simulink model "TwoSpeed_harness"  (Simulink 7.7)
settings: Solver=ode3  SolverMode=SingleTasking  StartTime=0.0  StopTime=100  FixedStep=.0005  RelTol=1e-3
PostLoadFcn:
  | cd '..';
  | PostLoadFcn;
  | cd 'harness';
InitFcn:
  | if signalbuilder('TwoSpeed_harness/Signal_Builder','activegroup') == 1
  |   CD_TWOSPEED_FUNCTION.DataType = 'uint8';
  |   CD_TWOSPEED_FUNCTION.Value = 255;
  | else
  |   CD_TWOSPEED_FUNCTION.DataType = 'uint8';
  |   CD_TWOSPEED_FUNCTION.Value = 0;
  | end
  | 
  | if signalbuilder('TwoSpeed_harness/Signal_Builder','activegroup') == 3
  |   CD_AUTOSHIFT_FUNCTION.DataType = 'uint8';
  |   CD_AUTOSHIFT_FUNCTION.Value = 0;
  |   CD_TWOSPEED_SWITCH_SOURCE.DataType = 'uint8';
  |   CD_TWOSPEED_SWITCH_SOURCE.Value = 23;
  | elseif signalbuilder('TwoSpeed_harness/Signal_Builder','activegroup') == 4
  |   CD_AUTOSHIFT_FUNCTION.DataType = 'uint8';
  |   CD_AUTOSHIFT_FUNCTION.Value = 0;
  |   CD_AUTOSHIFT_TRAVEL_DELAY.DataType = 'uint8';
  |   CD_AUTOSHIFT_TRAVEL_DELAY.Value = 0;
  | else
  |   CD_AUTOSHIFT_FUNCTION.DataType = 'uint8';
  |   CD_AUTOSHIFT_FUNCTION.Value = 255;
  |   CD_TWOSPEED_SWITCH_SOURCE.DataType = 'uint8';
  |   CD_TWOSPEED_SWITCH_SOURCE.Value = 176;
  |   CD_AUTOSHIFT_TRAVEL_DELAY.DataType = 'uint8';
  |   CD_AUTOSHIFT_TRAVEL_DELAY.Value = 32;
  | end
undefined symbols (not defined in the file): ACTIVE, CD_AUTOSHIFT_PHIGH1, CD_AUTOSHIFT_PHIGH2, CD_AUTOSHIFT_PHIGH_TEMP1, CD_AUTOSHIFT_PHIGH_TEMP2, CD_AUTOSHIFT_PLOW1, CD_AUTOSHIFT_PLOW2, CD_AUTOSHIFT_PLOW_TEMP1, CD_AUTOSHIFT_PLOW_TEMP2, CD_PRECISION_REF_NOMINAL_VALUE, CD_TWOSPEED_AFBK_GAIN, CD_TWOSPEED_DEBOUNCE_OPEN_CIRCUIT, CD_TWOSPEED_DEBOUNCE_SHORT_TO_BATTERY, CD_TWOSPEED_DEBOUNCE_SHORT_TO_GROUND, CD_VBATTERY_FILTER_DISPLAY_GAIN, CD_VBATTERY_FILTER_GAIN, CD_VBATTERY_GAIN, ENGINE_CRANKING, EXTREMELY_HIGH, FULL_ON, HIGH, INACTIVE, LOW, NON_FUNCTIONAL, NORMAL, OORH, OORL, SA_GATEWAY, sigbuilder_block, srate, srate100, SYS_NORMAL
libraries: simulink x12, MX_Library x1
settings Model: Creator=smindema  LastModifiedBy=aliebel  CovPath=Aux_Hydraulics/Aux_Hydraulics  CovMetricSettings=dcmw  CovHTMLOptions=-aTS=1 -bRG=1 -bTC=1 -hTR=0 -nFC=0 -scm=1 -bcm=1 -xEv=0  covSaveCumulativeToWorkspaceVar=off  CovSaveSingleToWorkspaceVar=off
settings MATStruct: SampleTime=0.01  Offset=0  Priority=[1.0]
settings DataIOCC: LimitDataPoints=off  SaveOutput=off  SaveTime=off
settings OptimizationCC: BlockReduction=off  InlineParams=on  ExpressionFolding=off  StateBitsets=on  DataBitsets=on  UseTempVars=on  InitFltsAndDblsToZero=on  NoFixptDivByZeroProtection=on  EfficientFloat2IntCast=on  OptimizeModelRefInitCode=on
settings DebuggingCC: SaveWithParameterizedLinksMsg=none  MultiTaskDSMMsg=warning  MultiTaskCondExecSysMsg=none  IntegerOverflowMsg=none  ModelReferenceCSMismatchMessage=warning
settings HardwareCC: ProdBitPerInt=16  ProdBitPerPointer=16  ProdIntDivRoundTo=Floor  ProdEndianess=BigEndian  ProdWordSize=16  ProdHWDeviceType=Motorola HC12
settings ModelReferenceCC: ModelReferenceNumInstancesAllowed=Single
settings RTWCC: SystemTargetFile=ert.tlc  GenCodeOnly=on  TemplateMakefile=ert_default_tmf  Description=Real-Time Workshop Embedded Coder (no auto configuration)  GenerateReport=on  RetainRTWFile=on  ProcessScript=ert_make_rtw_hook  IncludeHyperlinkInReport=on  LaunchReport=on  IncludeERTFirstTime=on
settings RTWCC: CustomHeaderCode=|
  | #include "cpp_req_defines.h"
  | #include "hw_fin.h"
  | #include "cdata.h"
settings CodeAppCC: IgnoreCustomStorageClasses=off  DefineNamingRule=UpperCase
settings ERTTargetCC: TargetFcnLib=ansi_tfl_tmw.mat  FunctionExecutionProfile=off  MultiwordLength=2048  GenerateSampleERTMain=on  IncludeMdlTerminateFcn=off  SupportAbsoluteTime=off  SupportNonFinite=off  SupportComplex=off  PurelyIntegerCode=on  ERTCustomFileTemplate=gen_rtw_req_defines_h.tlc  GlobalDataDefinition=InSeparateSourceFile  GlobalDataReference=InSeparateHeaderFile  ConvertIfToSwitch=off

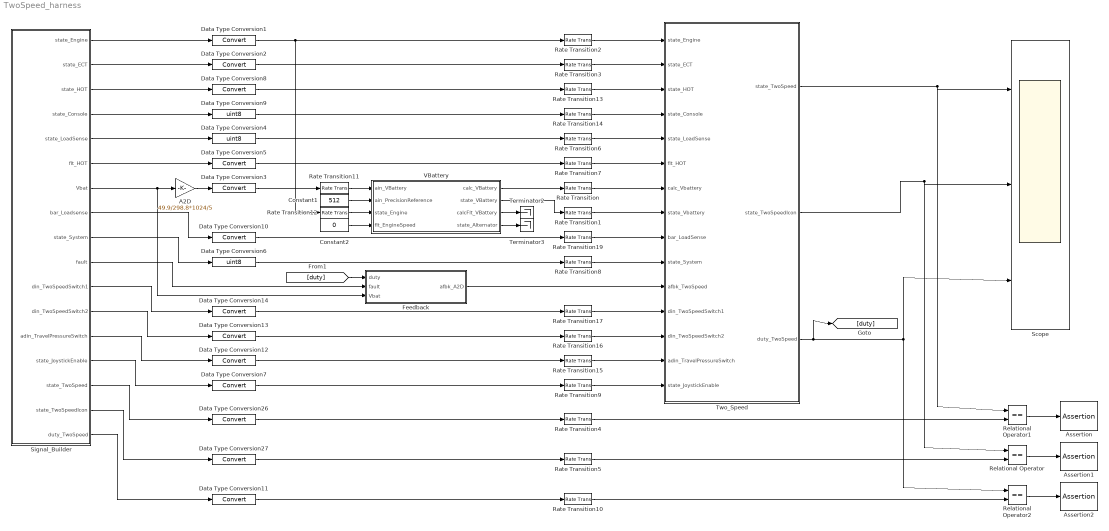
== system TwoSpeed_harness ==
  A2D : Gain  Gain=49.9/298.8*1024/5  OutDataTypeStr=uint16
  Assertion : Assertion  Enabled=off
  Assertion1 : Assertion  Enabled=off
  Assertion2 : Assertion  Enabled=off
  Constant1 : Constant  Value=512  OutDataTypeStr=uint16
  Constant2 : Constant  Value=0  OutDataTypeStr=uint16
  Data Type Conversion{1..3,5,7..8,10..14,26..27} (13 alike) : DataTypeConversion
  Data Type Conversion4 : DataTypeConversion  OutDataTypeStr=uint8
  Data Type Conversion6 : DataTypeConversion  OutDataTypeStr=uint8
  Data Type Conversion9 : DataTypeConversion  OutDataTypeStr=uint8
  Feedback : Subsystem
  Rate Transition : RateTransition  X0=12
  Rate Transition1 : RateTransition  X0=8
  Rate Transition{2..17,19} (17 alike) : RateTransition
  Relational Operator : RelationalOperator  Operator===  OutDataTypeStr=boolean
  Relational Operator1 : RelationalOperator  Operator===  OutDataTypeStr=boolean
  Relational Operator2 : RelationalOperator  Operator===  OutDataTypeStr=boolean
  Scope : Scope  NumInputPorts=3
      settings: TimeRange=50  YMin=0~0~0  YMax=0.3~1~1.25  DataFormat=Array
  Signal_Builder : Subsystem  Tag=STV Subsys  LoadFcn=sigbuilder_block('load');  StartFcn=sigbuilder_block('start');  StopFcn=sigbuilder_block('stop');  ClipboardFcn=sigbuilder_block('clipboard');  mask(Sigbuilder block){}
      mask help: Sigbuilder GUI
      mask init:
      | if ~strcmp(get_param(bdroot(gcbh),'SimulationStatus'),'stopped') tuvar = sigbuilder_block('maskInit'); end
      settings: CopyFcn=sigbuilder_block('copy');  DeleteFcn=sigbuilder_block('delete');  ModelCloseFcn=sigbuilder_block('modelClose');  PreSaveFcn=sigbuilder_block('preSave');  NameChangeFcn=sigbuilder_block('namechange');  OpenFcn=sigbuilder_block('open',[202.5 108.75 780.75 697.5 ]);  CloseFcn=sigbuilder_block('close');
      mask Display: plot(0,0,100,100,[10,10,40,40,10],[80,20,20,80,80],[40,10],[50,50], [40,27,10],[65,72,56],[40,25,25,10],[28,28,43,43]);
  Terminator2 : Terminator
  Terminator3 : Terminator
  Two_Speed : Subsystem  TreatAsAtomicUnit=on  SystemSampleTime=srate  RTWFileName=mod_Outputs
      settings: RTWSystemCode=Function  RTWFcnNameOpts=Use subsystem name  RTWFileNameOpts=User specified
  VBattery : Subsystem  TreatAsAtomicUnit=on  SystemSampleTime=srate100  RTWFileName=mod_Inputs
      settings: RTWSystemCode=Function  RTWFcnNameOpts=Use subsystem name  RTWFileNameOpts=User specified
  wires:
  Signal_Builder/2(state_ECT) -> Data Type Conversion2/1
  Relational Operator/1 -> Assertion1/1
  Signal_Builder/1(state_Engine) -> Data Type Conversion1/1
  Signal_Builder/5(state_LoadSense) -> Data Type Conversion4/1
  Relational Operator1/1 -> Assertion/1
  Data Type Conversion26/1 -> Rate Transition4/1
  Data Type Conversion27/1 -> Rate Transition5/1
  Data Type Conversion1/1 -> Rate Transition2/1, Rate Transition12/1
  Data Type Conversion2/1 -> Rate Transition3/1
  Data Type Conversion4/1 -> Rate Transition6/1
  Data Type Conversion5/1 -> Rate Transition7/1
  Data Type Conversion6/1 -> Rate Transition8/1
  Data Type Conversion7/1 -> Rate Transition9/1
  Signal_Builder/6(flt_HOT) -> Data Type Conversion5/1
  Signal_Builder/9(state_System) -> Data Type Conversion6/1
  VBattery/2(state_VBattery) -> Rate Transition1/1
  VBattery/1(calc_VBattery) -> Rate Transition/1
  VBattery/3(calcFlt_VBattery) -> Terminator2/1
  VBattery/4(state_Alternator) -> Terminator3/1
  Constant2/1 -> VBattery/4(flt_EngineSpeed)
  Signal_Builder/7(Vbat) -> Feedback/3(Vbat), A2D/1
  A2D/1 -> Data Type Conversion3/1
  Data Type Conversion3/1 -> Rate Transition11/1
  Signal_Builder/10(fault) -> Feedback/2(fault)
  [duty] -> Feedback/1(duty)
  Rate Transition1/1 -> Two_Speed/8(state_Vbattery)
  Rate Transition/1 -> Two_Speed/7(calc_Vbattery)
  Rate Transition2/1 -> Two_Speed/1(state_Engine)
  Rate Transition3/1 -> Two_Speed/2(state_ECT)
  Rate Transition4/1 -> Relational Operator1/2
  Rate Transition5/1 -> Relational Operator/2
  Rate Transition6/1 -> Two_Speed/5(state_LoadSense)
  Rate Transition7/1 -> Two_Speed/6(flt_HOT)
  Rate Transition8/1 -> Two_Speed/10(state_System)
  Rate Transition9/1 -> Two_Speed/15(state_JoystickEnable)
  Constant1/1 -> VBattery/2(ain_PrecisionReference)
  Rate Transition11/1 -> VBattery/1(ain_VBattery)
  Rate Transition12/1 -> VBattery/3(state_Engine)
  Feedback/1(afbk_A2D) -> Two_Speed/11(afbk_TwoSpeed)
  Signal_Builder/3(state_HOT) -> Data Type Conversion8/1
  Signal_Builder/4(state_Console) -> Data Type Conversion9/1
  Data Type Conversion8/1 -> Rate Transition13/1
  Data Type Conversion9/1 -> Rate Transition14/1
  Rate Transition13/1 -> Two_Speed/3(state_HOT)
  Rate Transition14/1 -> Two_Speed/4(state_Console)
  Signal_Builder/8(bar_Loadsense) -> Data Type Conversion10/1
  Data Type Conversion10/1 -> Rate Transition19/1
  Two_Speed/1(state_TwoSpeed) -> Scope/1, Relational Operator1/1
  Two_Speed/2(state_TwoSpeedIcon) -> Scope/2, Relational Operator/1
  Two_Speed/3(duty_TwoSpeed) -> [duty], Scope/3, Relational Operator2/1
  Relational Operator2/1 -> Assertion2/1
  Data Type Conversion11/1 -> Rate Transition10/1
  Rate Transition10/1 -> Relational Operator2/2
  Signal_Builder/11(din_TwoSpeedSwitch1) -> Data Type Conversion14/1
  Signal_Builder/12(din_TwoSpeedSwitch2) -> Data Type Conversion13/1
  Signal_Builder/13(adin_TravelPressureSwitch) -> Data Type Conversion12/1
  Signal_Builder/14(state_JoystickEnable) -> Data Type Conversion7/1
  Signal_Builder/15(state_TwoSpeed) -> Data Type Conversion26/1
  Signal_Builder/16(state_TwoSpeedIcon) -> Data Type Conversion27/1
  Signal_Builder/17(duty_TwoSpeed) -> Data Type Conversion11/1
  Data Type Conversion12/1 -> Rate Transition15/1
  Data Type Conversion13/1 -> Rate Transition16/1
  Data Type Conversion14/1 -> Rate Transition17/1
  Rate Transition15/1 -> Two_Speed/14(adin_TravelPressureSwitch)
  Rate Transition16/1 -> Two_Speed/13(din_TwoSpeedSwitch2)
  Rate Transition17/1 -> Two_Speed/12(din_TwoSpeedSwitch1)
  Rate Transition19/1 -> Two_Speed/9(bar_LoadSense)

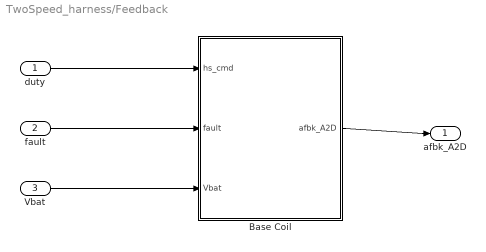
== system TwoSpeed_harness/Feedback ==
  duty : Inport
  fault : Inport  Port=2
  Vbat : Inport  Port=3
  Base Coil : Subsystem
  afbk_A2D : Outport
  wires:
  Base Coil/1(afbk_A2D) -> afbk_A2D/1
  duty/1 -> Base Coil/1(hs_cmd)
  fault/1 -> Base Coil/2(fault)
  Vbat/1 -> Base Coil/3(Vbat)

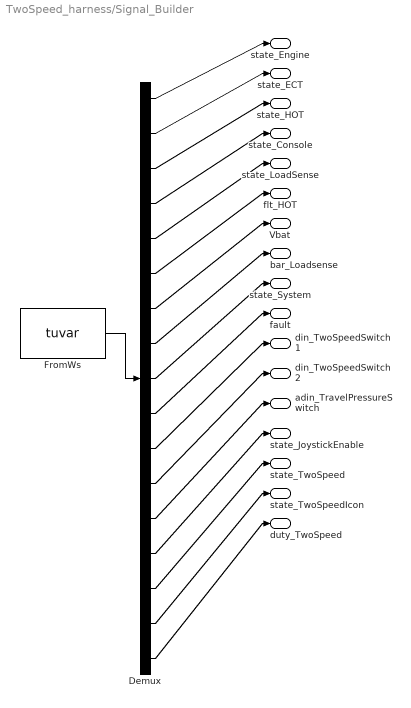
== system TwoSpeed_harness/Signal_Builder ==
  Demux : Demux  Tag=STV Demux  Outputs=17
  FromWs : FromWorkspace  Tag=STV FromWs  VariableName=tuvar  SampleTime=0  SigBuilderData=DataTag0  VnvData=DataTag1
      SigBuilderData=|
      | common.afterFinalStr = 'Extrapolate'
      | common.sampleTime = 0
      | dataSet(1).timeRange = [0 100]
      | dataSet(1).name = 'NonFunctional'
      | dataSet(2).timeRange = [0 100]
      | dataSet(2).name = 'Functional - Normal'
      | dataSet(3).timeRange = [0 100]
      | dataSet(3).name = 'Functional - Autoshift'
      | dataSet(4).timeRange = [0 100]
      | dataSet(4).name = 'Functional - Autoshift1'
      | dataSet(5).timeRange = [0 100]
      | dataSet(5).name = 'STB'
      | dataSet(6).timeRange = [0 100]
      | dataSet(6).name = 'STG'
      | dataSet(7).timeRange = [0 100]
      | dataSet(7).name = 'Open'
      | sbobj.Groups(1).Name = 'NonFunctional'
      | sbobj.Groups(1).Signals(1).Name = 'state_Engine'
      | sbobj.Groups(1).Signals(1).XData = [0 24 24 26 26 37 37 39 39 77 82 100]
      | sbobj.Groups(1).Signals(1).YData = [0 0 2 2 0 0 2 2 0 0 0 0]
      | sbobj.Groups(1).Signals(2).Name = 'state_ECT'
      | sbobj.Groups(1).Signals(2).XData = [0 10 10 11 11 12 12 20 20 21 21 22 22 23 23 48 52 100]
      | sbobj.Groups(1).Signals(2).YData = [8 8 10 10 11 11 8 8 10 10 8 8 11 11 8 8 8 8]
      | sbobj.Groups(1).Signals(3).Name = 'state_HOT'
      | sbobj.Groups(1).Signals(3).XData = [0 6 6 8 8 9 9 16 16 17 17 18 18 19 19 49.4 53.6 56.6 61 100]
      | sbobj.Groups(1).Signals(3).YData = [8 8 10 10 11 11 8 8 10 10 8 8 11 11 8 8 8 8 8 8]
      | sbobj.Groups(1).Signals(4).Name = 'state_Console'
      | sbobj.Groups(1).Signals(4).XData = [0 1 1 5 5 7 7 64.8 64.8 100]
      | sbobj.Groups(1).Signals(4).YData = [0 0 1 1 0 0 1 1 0 0]
      | sbobj.Groups(1).Signals(5).Name = 'state_LoadSense'
      | sbobj.Groups(1).Signals(5).XData = [0 100]
      | sbobj.Groups(1).Signals(5).YData = [8 8]
      | sbobj.Groups(1).Signals(6).Name = 'flt_HOT'
      | sbobj.Groups(1).Signals(6).XData = [0 100]
      | sbobj.Groups(1).Signals(6).YData = [110 110]
      | sbobj.Groups(1).Signals(7).Name = 'Vbat'
      | sbobj.Groups(1).Signals(7).XData = [0 100]
      | sbobj.Groups(1).Signals(7).YData = [12 12]
      | sbobj.Groups(1).Signals(8).Name = 'bar_Loadsense'
      | sbobj.Groups(1).Signals(8).XData = [0 100]
      | sbobj.Groups(1).Signals(8).YData = [0 0]
      | sbobj.Groups(1).Signals(9).Name = 'state_System'
      | sbobj.Groups(1).Signals(9).XData = [0 90 90 100]
      | sbobj.Groups(1).Signals(9).YData = [1 1 2 2]
      | sbobj.Groups(1).Signals(10).Name = 'fault'
      | sbobj.Groups(1).Signals(10).XData = [0 100]
      | sbobj.Groups(1).Signals(10).YData = [0 0]
      | sbobj.Groups(1).Signals(11).Name = 'din_TwoSpeedSwitch1'
      | sbobj.Groups(1).Signals(11).XData = [0 2 2 2.5 2.5 4 4 4.5 4.5 13 13 13.5 13.5 25 25 25.5 25.5 100]
      | sbobj.Groups(1).Signals(11).YData = [0 0 1 1 0 0 1 1 0 0 1 1 0 0 1 1 0 0]
      | sbobj.Groups(1).Signals(12).Name = 'din_TwoSpeedSwitch2'
      | sbobj.Groups(1).Signals(12).XData = [0 40 53 100]
      | sbobj.Groups(1).Signals(12).YData = [0 0 0 0]
      | sbobj.Groups(1).Signals(13).Name = 'adin_TravelPressureSwitch'
      | sbobj.Groups(1).Signals(13).XData = [0 100]
      | sbobj.Groups(1).Signals(13).YData = [0 0]
      | sbobj.Groups(1).Signals(14).Name = 'state_JoystickEnable'
      | sbobj.Groups(1).Signals(14).XData = [0 24 24 28 28 32 32 35 35 100]
      | sbobj.Groups(1).Signals(14).YData = [1 1 0 0 1 1 0 0 1 1]
      | sbobj.Groups(1).Signals(15).Name = 'state_TwoSpeed'
      | sbobj.Groups(1).Signals(15).XData = [0 100]
      | sbobj.Groups(1).Signals(15).YData = [0 0]
      | sbobj.Groups(1).Signals(16).Name = 'state_TwoSpeedIcon'
      | sbobj.Groups(1).Signals(16).XData = [0 100]
      | sbobj.Groups(1).Signals(16).YData = [0 0]
      | sbobj.Groups(1).Signals(17).Name = 'duty_TwoSpeed'
      | sbobj.Groups(1).Signals(17).XData = [0 100]
      | sbobj.Groups(1).Signals(17).YData = [0 0]
      | sbobj.Groups(1).TimeRange = [0 100]
      | sbobj.Groups(2).Name = 'Functional - Normal'
      | sbobj.Groups(2).Signals(1).Name = 'state_Engine'
      | sbobj.Groups(2).Signals(1).XData = [0 24 24 26 26 37 37 39 39 77 82 100]
      | sbobj.Groups(2).Signals(1).YData = [0 0 2 2 0 0 2 2 0 0 0 0]
      | sbobj.Groups(2).Signals(2).Name = 'state_ECT'
      | sbobj.Groups(2).Signals(2).XData = [0 10 10 11 11 12 12 20 20 21 21 22 22 23 23 48 52 100]
      | sbobj.Groups(2).Signals(2).YData = [8 8 10 10 11 11 8 8 10 10 8 8 11 11 8 8 8 8]
      | sbobj.Groups(2).Signals(3).Name = 'state_HOT'
      | sbobj.Groups(2).Signals(3).XData = [0 6 6 8 8 9 9 16 16 17 17 18 18 19 19 49.4 53.6 56.6 61 100]
      | sbobj.Groups(2).Signals(3).YData = [8 8 10 10 11 11 8 8 10 10 8 8 11 11 8 8 8 8 8 8]
      | sbobj.Groups(2).Signals(4).Name = 'state_Console'
      | sbobj.Groups(2).Signals(4).XData = [0 1 1 5 5 7 7 64.8 64.8 100]
      | sbobj.Groups(2).Signals(4).YData = [0 0 1 1 0 0 1 1 0 0]
      | sbobj.Groups(2).Signals(5).Name = 'state_LoadSense'
      | sbobj.Groups(2).Signals(5).XData = [0 100]
      | sbobj.Groups(2).Signals(5).YData = [8 8]
      | sbobj.Groups(2).Signals(6).Name = 'flt_HOT'
      | sbobj.Groups(2).Signals(6).XData = [0 100]
      | sbobj.Groups(2).Signals(6).YData = [110 110]
      | sbobj.Groups(2).Signals(7).Name = 'Vbat'
      | sbobj.Groups(2).Signals(7).XData = [0 100]
      | sbobj.Groups(2).Signals(7).YData = [12 12]
      | sbobj.Groups(2).Signals(8).Name = 'bar_Loadsense'
      | sbobj.Groups(2).Signals(8).XData = [0 100]
      | sbobj.Groups(2).Signals(8).YData = [0 0]
      | sbobj.Groups(2).Signals(9).Name = 'state_System'
      | sbobj.Groups(2).Signals(9).XData = [0 90 90 100]
      | sbobj.Groups(2).Signals(9).YData = [1 1 2 2]
      | sbobj.Groups(2).Signals(10).Name = 'fault'
      | sbobj.Groups(2).Signals(10).XData = [0 100]
      | sbobj.Groups(2).Signals(10).YData = [0 0]
      | sbobj.Groups(2).Signals(11).Name = 'din_TwoSpeedSwitch1'
      | sbobj.Groups(2).Signals(11).XData = [0 2 2 2.5 2.5 4 4 4.5 4.5 13 13 13.5 13.5 25 25 25.5 25.5 100]
      | sbobj.Groups(2).Signals(11).YData = [0 0 1 1 0 0 1 1 0 0 1 1 0 0 1 1 0 0]
      | sbobj.Groups(2).Signals(12).Name = 'din_TwoSpeedSwitch2'
      | sbobj.Groups(2).Signals(12).XData = [0 40 53 100]
      | sbobj.Groups(2).Signals(12).YData = [0 0 0 0]
      | sbobj.Groups(2).Signals(13).Name = 'adin_TravelPressureSwitch'
      | sbobj.Groups(2).Signals(13).XData = [0 100]
      | sbobj.Groups(2).Signals(13).YData = [0 0]
      | sbobj.Groups(2).Signals(14).Name = 'state_JoystickEnable'
      | sbobj.Groups(2).Signals(14).XData = [0 24 24 28 28 32 32 35 35 100]
      | sbobj.Groups(2).Signals(14).YData = [1 1 0 0 1 1 0 0 1 1]
      | sbobj.Groups(2).Signals(15).Name = 'state_TwoSpeed'
      | sbobj.Groups(2).Signals(15).XData = [0 100]
      | sbobj.Groups(2).Signals(15).YData = [0 0]
      | sbobj.Groups(2).Signals(16).Name = 'state_TwoSpeedIcon'
      | sbobj.Groups(2).Signals(16).XData = [0 100]
      | sbobj.Groups(2).Signals(16).YData = [0 0]
      | sbobj.Groups(2).Signals(17).Name = 'duty_TwoSpeed'
      | sbobj.Groups(2).Signals(17).XData = [0 100]
      | sbobj.Groups(2).Signals(17).YData = [0 0]
      | sbobj.Groups(2).TimeRange = [0 100]
      | sbobj.Groups(3).Name = 'Functional - Autoshift'
      | sbobj.Groups(3).Signals(1).Name = 'state_Engine'
      | sbobj.Groups(3).Signals(1).XData = [0 24 24 26 26 37 37 39 39 77 82 100]
      | sbobj.Groups(3).Signals(1).YData = [0 0 2 2 0 0 2 2 0 0 0 0]
      | sbobj.Groups(3).Signals(2).Name = 'state_ECT'
      | sbobj.Groups(3).Signals(2).XData = [0 10 10 11 11 12 12 20 20 21 21 22 22 23 23 48 52 100]
      | sbobj.Groups(3).Signals(2).YData = [8 8 10 10 11 11 8 8 10 10 8 8 11 11 8 8 8 8]
      | sbobj.Groups(3).Signals(3).Name = 'state_HOT'
      | sbobj.Groups(3).Signals(3).XData = [0 6 6 8 8 9 9 16 16 17 17 18 18 19 19 49.4 53.6 56.6 61 100]
      | sbobj.Groups(3).Signals(3).YData = [8 8 10 10 11 11 8 8 10 10 8 8 11 11 8 8 8 8 8 8]
      | sbobj.Groups(3).Signals(4).Name = 'state_Console'
      | sbobj.Groups(3).Signals(4).XData = [0 1 1 5 5 7 7 63.8 63.8 65.2 65.2 70.2 70.2 71.4 71.4 74 74 75 75 83.4 83.4 84.4 84.4 100]
      | sbobj.Groups(3).Signals(4).YData = [0 0 1 1 0 0 1 1 0 0 1 1 0 0 1 1 0 0 1 1 0 0 1 1]
      | sbobj.Groups(3).Signals(5).Name = 'state_LoadSense'
      | sbobj.Groups(3).Signals(5).XData = [0 52 52 54 54 55 55 57 57 100]
      | sbobj.Groups(3).Signals(5).YData = [8 8 21 21 8 8 21 21 8 8]
      | sbobj.Groups(3).Signals(6).Name = 'flt_HOT'
      | sbobj.Groups(3).Signals(6).XData = [0 100]
      | sbobj.Groups(3).Signals(6).YData = [110 110]
      | sbobj.Groups(3).Signals(7).Name = 'Vbat'
      | sbobj.Groups(3).Signals(7).XData = [0 100]
      | sbobj.Groups(3).Signals(7).YData = [12 12]
      | sbobj.Groups(3).Signals(8).Name = 'bar_Loadsense'
      | sbobj.Groups(3).Signals(8).XData = [0 42 42 50 50 53 53 59 59 82 82 100]
      | sbobj.Groups(3).Signals(8).YData = [0 0 207 207 95 95 210 210 95 95 210 210]
      | sbobj.Groups(3).Signals(9).Name = 'state_System'
      | sbobj.Groups(3).Signals(9).XData = [0 97 97 100]
      | sbobj.Groups(3).Signals(9).YData = [1 1 2 2]
      | sbobj.Groups(3).Signals(10).Name = 'fault'
      | sbobj.Groups(3).Signals(10).XData = [0 100]
      | sbobj.Groups(3).Signals(10).YData = [0 0]
      | sbobj.Groups(3).Signals(11).Name = 'din_TwoSpeedSwitch1'
      | sbobj.Groups(3).Signals(11).XData = [0 100]
      | sbobj.Groups(3).Signals(11).YData = [0 0]
      | sbobj.Groups(3).Signals(12).Name = 'din_TwoSpeedSwitch2'
      | sbobj.Groups(3).Signals(12).XData = [0 2 2 3 3 4 4 5 5 13 13 14 14 25 25 26 26 67 67 68 68 73 73 74 74 78 78 79 79 100]
      | sbobj.Groups(3).Signals(12).YData = [0 0 1 1 0 0 1 1 0 0 1 1 0 0 1 1 0 0 1 1 0 0 1 1 0 0 1 1 0 0]
      | sbobj.Groups(3).Signals(13).Name = 'adin_TravelPressureSwitch'
      | sbobj.Groups(3).Signals(13).XData = [0 40.2 40.2 44 44 46 46 48 48 49.4 49.4 60 60 61 61 61.2 61.2 70 70 88.2 88.2 100]
      | sbobj.Groups(3).Signals(13).YData = [0 0 1023 1023 0 0 1023 1023 0 0 1023 1023 0 0 1023 1023 0 0 1023 1023 0 0]
      | sbobj.Groups(3).Signals(14).Name = 'state_JoystickEnable'
      | sbobj.Groups(3).Signals(14).XData = [0 24 24 28 28 32 32 35 35 100]
      | sbobj.Groups(3).Signals(14).YData = [1 1 0 0 1 1 0 0 1 1]
      | sbobj.Groups(3).Signals(15).Name = 'state_TwoSpeed'
      | sbobj.Groups(3).Signals(15).XData = [0 100]
      | sbobj.Groups(3).Signals(15).YData = [0 0]
      | sbobj.Groups(3).Signals(16).Name = 'state_TwoSpeedIcon'
      | sbobj.Groups(3).Signals(16).XData = [0 100]
      | sbobj.Groups(3).Signals(16).YData = [0 0]
      | sbobj.Groups(3).Signals(17).Name = 'duty_TwoSpeed'
      | sbobj.Groups(3).Signals(17).XData = [0 100]
      | sbobj.Groups(3).Signals(17).YData = [0 0]
      | sbobj.Groups(3).TimeRange = [0 100]
      | sbobj.Groups(4).Name = 'Functional - Autoshift1'
      | sbobj.Groups(4).Signals(1).Name = 'state_Engine'
      | sbobj.Groups(4).Signals(1).XData = [0 24 24 26 26 37 37 39 39 77 82 100]
      | sbobj.Groups(4).Signals(1).YData = [0 0 2 2 0 0 2 2 0 0 0 0]
      | sbobj.Groups(4).Signals(2).Name = 'state_ECT'
      | sbobj.Groups(4).Signals(2).XData = [0 10 10 11 11 12 12 20 20 21 21 22 22 23 23 48 52 52 100]
      | sbobj.Groups(4).Signals(2).YData = [8 8 10 10 11 11 8 8 10 10 8 8 11 11 8 8 8 8 8]
      | sbobj.Groups(4).Signals(3).Name = 'state_HOT'
      | sbobj.Groups(4).Signals(3).XData = [0 6 6 8 8 9 9 16 16 17 17 18 18 19 19 93 93 93.6 93.6 95 95 95.8 95.8 100]
      | sbobj.Groups(4).Signals(3).YData = [8 8 10 10 11 11 8 8 10 10 8 8 11 11 8 8 21 21 8 8 22 22 8 8]
      | sbobj.Groups(4).Signals(4).Name = 'state_Console'
      | sbobj.Groups(4).Signals(4).XData = [0 1 1 5 5 7 7 63.8 63.8 65.2 65.2 70.2 70.2 71.4 71.4 74 74 75 75 83.4 83.4 84.4 84.4 100]
      | sbobj.Groups(4).Signals(4).YData = [0 0 1 1 0 0 1 1 0 0 1 1 0 0 1 1 0 0 1 1 0 0 1 1]
      | sbobj.Groups(4).Signals(5).Name = 'state_LoadSense'
      | sbobj.Groups(4).Signals(5).XData = [0 52 52 54 54 55 55 57 57 100]
      | sbobj.Groups(4).Signals(5).YData = [8 8 21 21 8 8 21 21 8 8]
      | sbobj.Groups(4).Signals(6).Name = 'flt_HOT'
      | sbobj.Groups(4).Signals(6).XData = [0 100]
      | sbobj.Groups(4).Signals(6).YData = [110 110]
      | sbobj.Groups(4).Signals(7).Name = 'Vbat'
      | sbobj.Groups(4).Signals(7).XData = [0 100]
      | sbobj.Groups(4).Signals(7).YData = [12 12]
      | sbobj.Groups(4).Signals(8).Name = 'bar_Loadsense'
      | sbobj.Groups(4).Signals(8).XData = [0 42 42 50 50 53 53 59 59 82 82 100]
      | sbobj.Groups(4).Signals(8).YData = [0 0 207 207 95 95 210 210 95 95 210 210]
      | sbobj.Groups(4).Signals(9).Name = 'state_System'
      | sbobj.Groups(4).Signals(9).XData = [0 97 97 100]
      | sbobj.Groups(4).Signals(9).YData = [1 1 2 2]
      | sbobj.Groups(4).Signals(10).Name = 'fault'
      | sbobj.Groups(4).Signals(10).XData = [0 100]
      | sbobj.Groups(4).Signals(10).YData = [0 0]
      | sbobj.Groups(4).Signals(11).Name = 'din_TwoSpeedSwitch1'
      | sbobj.Groups(4).Signals(11).XData = [0 100]
      | sbobj.Groups(4).Signals(11).YData = [0 0]
      | sbobj.Groups(4).Signals(12).Name = 'din_TwoSpeedSwitch2'
      | sbobj.Groups(4).Signals(12).XData = [0 2 2 3 3 4 4 5 5 13 13 14 14 25 25 26 26 67 67 68 68 73 73 74 74 78 78 79 79 100]
      | sbobj.Groups(4).Signals(12).YData = [0 0 1 1 0 0 1 1 0 0 1 1 0 0 1 1 0 0 1 1 0 0 1 1 0 0 1 1 0 0]
      | sbobj.Groups(4).Signals(13).Name = 'adin_TravelPressureSwitch'
      | sbobj.Groups(4).Signals(13).XData = [0 40.2 40.2 44 44 46 46 48 48 49.4 49.4 60 60 61 61 61.2 61.2 70 70 95.6 95.6 100]
      | sbobj.Groups(4).Signals(13).YData = [0 0 1023 1023 0 0 1023 1023 0 0 1023 1023 0 0 1023 1023 0 0 1023 1023 0 0]
      | sbobj.Groups(4).Signals(14).Name = 'state_JoystickEnable'
      | sbobj.Groups(4).Signals(14).XData = [0 24 24 28 28 32 32 35 35 100]
      | sbobj.Groups(4).Signals(14).YData = [1 1 0 0 1 1 0 0 1 1]
      | sbobj.Groups(4).Signals(15).Name = 'state_TwoSpeed'
      | sbobj.Groups(4).Signals(15).XData = [0 100]
      | sbobj.Groups(4).Signals(15).YData = [0 0]
      | sbobj.Groups(4).Signals(16).Name = 'state_TwoSpeedIcon'
      | sbobj.Groups(4).Signals(16).XData = [0 100]
      | sbobj.Groups(4).Signals(16).YData = [0 0]
      | sbobj.Groups(4).Signals(17).Name = 'duty_TwoSpeed'
      | sbobj.Groups(4).Signals(17).XData = [0 100]
      | sbobj.Groups(4).Signals(17).YData = [0 0]
      | sbobj.Groups(4).TimeRange = [0 100]
      | sbobj.Groups(5).Name = 'STB'
      | sbobj.Groups(5).Signals(1).Name = 'state_Engine'
      | sbobj.Groups(5).Signals(1).XData = [0 50 50 54 54 100]
      | sbobj.Groups(5).Signals(1).YData = [0 0 2 2 0 0]
      | sbobj.Groups(5).Signals(2).Name = 'state_ECT'
      | sbobj.Groups(5).Signals(2).XData = [0 100]
      | sbobj.Groups(5).Signals(2).YData = [8 8]
      | sbobj.Groups(5).Signals(3).Name = 'state_HOT'
      | sbobj.Groups(5).Signals(3).XData = [0 100]
      | sbobj.Groups(5).Signals(3).YData = [8 8]
      | sbobj.Groups(5).Signals(4).Name = 'state_Console'
      | sbobj.Groups(5).Signals(4).XData = [0 15.8 15.8 100]
      | sbobj.Groups(5).Signals(4).YData = [0 0 1 1]
      | sbobj.Groups(5).Signals(5).Name = 'state_LoadSense'
      | sbobj.Groups(5).Signals(5).XData = [0 100]
      | sbobj.Groups(5).Signals(5).YData = [8 8]
      | sbobj.Groups(5).Signals(6).Name = 'flt_HOT'
      | sbobj.Groups(5).Signals(6).XData = [0 100]
      | sbobj.Groups(5).Signals(6).YData = [110 110]
      | sbobj.Groups(5).Signals(7).Name = 'Vbat'
      | sbobj.Groups(5).Signals(7).XData = [0 50 50 58 58 100]
      | sbobj.Groups(5).Signals(7).YData = [12 12 5 5 12 12]
      | sbobj.Groups(5).Signals(8).Name = 'bar_Loadsense'
      | sbobj.Groups(5).Signals(8).XData = [0 100]
      | sbobj.Groups(5).Signals(8).YData = [0 0]
      | sbobj.Groups(5).Signals(9).Name = 'state_System'
      | sbobj.Groups(5).Signals(9).XData = [0 12 12 13 13 37 37 38 38 100]
      | sbobj.Groups(5).Signals(9).YData = [1 1 2 2 1 1 2 2 1 1]
      | sbobj.Groups(5).Signals(10).Name = 'fault'
      | sbobj.Groups(5).Signals(10).XData = [0 4 4 4.02 4.02 5.73 5.73 7.65 7.65 22 22 22.02 22.02 25.48 25.48 27.79 27.79 100]
      | sbobj.Groups(5).Signals(10).YData = [0 0 1 1 0 0 1 1 0 0 1 1 0 0 1 1 0 0]
      | sbobj.Groups(5).Signals(11).Name = 'din_TwoSpeedSwitch1'
      | sbobj.Groups(5).Signals(11).XData = [0 18 18 19 19 100]
      | sbobj.Groups(5).Signals(11).YData = [0 0 1 1 0 0]
      | sbobj.Groups(5).Signals(12).Name = 'din_TwoSpeedSwitch2'
      | sbobj.Groups(5).Signals(12).XData = [0 40 53 100]
      | sbobj.Groups(5).Signals(12).YData = [0 0 0 0]
      | sbobj.Groups(5).Signals(13).Name = 'adin_TravelPressureSwitch'
      | sbobj.Groups(5).Signals(13).XData = [0 100]
      | sbobj.Groups(5).Signals(13).YData = [0 0]
      | sbobj.Groups(5).Signals(14).Name = 'state_JoystickEnable'
      | sbobj.Groups(5).Signals(14).XData = [0 100]
      | sbobj.Groups(5).Signals(14).YData = [1 1]
      | sbobj.Groups(5).Signals(15).Name = 'state_TwoSpeed'
      | sbobj.Groups(5).Signals(15).XData = [0 100]
      | sbobj.Groups(5).Signals(15).YData = [0 0]
      | sbobj.Groups(5).Signals(16).Name = 'state_TwoSpeedIcon'
      | sbobj.Groups(5).Signals(16).XData = [0 100]
      | sbobj.Groups(5).Signals(16).YData = [0 0]
      | sbobj.Groups(5).Signals(17).Name = 'duty_TwoSpeed'
      | sbobj.Groups(5).Signals(17).XData = [0 100]
      | sbobj.Groups(5).Signals(17).YData = [0 0]
      | sbobj.Groups(5).TimeRange = [0 100]
      | sbobj.Groups(6).Name = 'STG'
      | sbobj.Groups(6).Signals(1).Name = 'state_Engine'
      | sbobj.Groups(6).Signals(1).XData = [0 50 50 54 54 100]
      | sbobj.Groups(6).Signals(1).YData = [0 0 2 2 0 0]
      | sbobj.Groups(6).Signals(2).Name = 'state_ECT'
      | sbobj.Groups(6).Signals(2).XData = [0 100]
      | sbobj.Groups(6).Signals(2).YData = [8 8]
      | sbobj.Groups(6).Signals(3).Name = 'state_HOT'
      | sbobj.Groups(6).Signals(3).XData = [0 100]
      | sbobj.Groups(6).Signals(3).YData = [8 8]
      | sbobj.Groups(6).Signals(4).Name = 'state_Console'
      | sbobj.Groups(6).Signals(4).XData = [0 15.8 15.8 100]
      | sbobj.Groups(6).Signals(4).YData = [0 0 1 1]
      | sbobj.Groups(6).Signals(5).Name = 'state_LoadSense'
      | sbobj.Groups(6).Signals(5).XData = [0 100]
      | sbobj.Groups(6).Signals(5).YData = [8 8]
      | sbobj.Groups(6).Signals(6).Name = 'flt_HOT'
      | sbobj.Groups(6).Signals(6).XData = [0 100]
      | sbobj.Groups(6).Signals(6).YData = [110 110]
      | sbobj.Groups(6).Signals(7).Name = 'Vbat'
      | sbobj.Groups(6).Signals(7).XData = [0 50 50 58 58 100]
      | sbobj.Groups(6).Signals(7).YData = [12 12 5 5 12 12]
      | sbobj.Groups(6).Signals(8).Name = 'bar_Loadsense'
      | sbobj.Groups(6).Signals(8).XData = [0 100]
      | sbobj.Groups(6).Signals(8).YData = [0 0]
      | sbobj.Groups(6).Signals(9).Name = 'state_System'
      | sbobj.Groups(6).Signals(9).XData = [0 12 12 13 13 37 37 38 38 100]
      | sbobj.Groups(6).Signals(9).YData = [1 1 2 2 1 1 2 2 1 1]
      | sbobj.Groups(6).Signals(10).Name = 'fault'
      | sbobj.Groups(6).Signals(10).XData = [0 4 4 4.02 4.02 5.73 5.73 7.65 7.65 22 22 22.02 22.02 25.48 25.48 27.79 27.79 48.05 53.06 100]
      | sbobj.Groups(6).Signals(10).YData = [0 0 2 2 0 0 2 2 0 0 2 2 0 0 2 2 0 0 0 0]
      | sbobj.Groups(6).Signals(11).Name = 'din_TwoSpeedSwitch1'
      | sbobj.Groups(6).Signals(11).XData = [0 18 18 19 19 100]
      | sbobj.Groups(6).Signals(11).YData = [0 0 1 1 0 0]
      | sbobj.Groups(6).Signals(12).Name = 'din_TwoSpeedSwitch2'
      | sbobj.Groups(6).Signals(12).XData = [0 40 53 100]
      | sbobj.Groups(6).Signals(12).YData = [0 0 0 0]
      | sbobj.Groups(6).Signals(13).Name = 'adin_TravelPressureSwitch'
      | sbobj.Groups(6).Signals(13).XData = [0 100]
      | sbobj.Groups(6).Signals(13).YData = [0 0]
      | sbobj.Groups(6).Signals(14).Name = 'state_JoystickEnable'
      | sbobj.Groups(6).Signals(14).XData = [0 100]
      | sbobj.Groups(6).Signals(14).YData = [1 1]
      | sbobj.Groups(6).Signals(15).Name = 'state_TwoSpeed'
      | sbobj.Groups(6).Signals(15).XData = [0 100]
      | sbobj.Groups(6).Signals(15).YData = [0 0]
      | sbobj.Groups(6).Signals(16).Name = 'state_TwoSpeedIcon'
      | sbobj.Groups(6).Signals(16).XData = [0 100]
      | sbobj.Groups(6).Signals(16).YData = [0 0]
      | sbobj.Groups(6).Signals(17).Name = 'duty_TwoSpeed'
      | sbobj.Groups(6).Signals(17).XData = [0 100]
      | sbobj.Groups(6).Signals(17).YData = [0 0]
      | sbobj.Groups(6).TimeRange = [0 100]
      | sbobj.Groups(7).Name = 'Open'
      | sbobj.Groups(7).Signals(1).Name = 'state_Engine'
      | sbobj.Groups(7).Signals(1).XData = [0 50 50 54 54 100]
      | sbobj.Groups(7).Signals(1).YData = [0 0 2 2 0 0]
      | sbobj.Groups(7).Signals(2).Name = 'state_ECT'
      | sbobj.Groups(7).Signals(2).XData = [0 100]
      | sbobj.Groups(7).Signals(2).YData = [8 8]
      | sbobj.Groups(7).Signals(3).Name = 'state_HOT'
      | sbobj.Groups(7).Signals(3).XData = [0 100]
      | sbobj.Groups(7).Signals(3).YData = [8 8]
      | sbobj.Groups(7).Signals(4).Name = 'state_Console'
      | sbobj.Groups(7).Signals(4).XData = [0 15.8 15.8 100]
      | sbobj.Groups(7).Signals(4).YData = [0 0 1 1]
      | sbobj.Groups(7).Signals(5).Name = 'state_LoadSense'
      | sbobj.Groups(7).Signals(5).XData = [0 100]
      | sbobj.Groups(7).Signals(5).YData = [8 8]
      | sbobj.Groups(7).Signals(6).Name = 'flt_HOT'
      | sbobj.Groups(7).Signals(6).XData = [0 100]
      | sbobj.Groups(7).Signals(6).YData = [110 110]
      | sbobj.Groups(7).Signals(7).Name = 'Vbat'
      | sbobj.Groups(7).Signals(7).XData = [0 50 50 58 58 100]
      | sbobj.Groups(7).Signals(7).YData = [12 12 5 5 12 12]
      | sbobj.Groups(7).Signals(8).Name = 'bar_Loadsense'
      | sbobj.Groups(7).Signals(8).XData = [0 100]
      | sbobj.Groups(7).Signals(8).YData = [0 0]
      | sbobj.Groups(7).Signals(9).Name = 'state_System'
      | sbobj.Groups(7).Signals(9).XData = [0 12 12 13 13 37 37 38 38 100]
      | sbobj.Groups(7).Signals(9).YData = [1 1 2 2 1 1 2 2 1 1]
      | sbobj.Groups(7).Signals(10).Name = 'fault'
      | sbobj.Groups(7).Signals(10).XData = [0 4 4 4.02 4.02 5.73 5.73 7.65 7.65 22 22 22.02 22.02 25.48 25.48 27.79 27.79 100]
      | sbobj.Groups(7).Signals(10).YData = [0 0 3 3 0 0 3 3 0 0 3 3 0 0 3 3 0 0]
      | sbobj.Groups(7).Signals(11).Name = 'din_TwoSpeedSwitch1'
      | sbobj.Groups(7).Signals(11).XData = [0 18 18 19 19 100]
      | sbobj.Groups(7).Signals(11).YData = [0 0 1 1 0 0]
      | sbobj.Groups(7).Signals(12).Name = 'din_TwoSpeedSwitch2'
      | sbobj.Groups(7).Signals(12).XData = [0 40 53 100]
      | sbobj.Groups(7).Signals(12).YData = [0 0 0 0]
      | sbobj.Groups(7).Signals(13).Name = 'adin_TravelPressureSwitch'
      | sbobj.Groups(7).Signals(13).XData = [0 100]
      | sbobj.Groups(7).Signals(13).YData = [0 0]
      | sbobj.Groups(7).Signals(14).Name = 'state_JoystickEnable'
      | sbobj.Groups(7).Signals(14).XData = [0 100]
      | sbobj.Groups(7).Signals(14).YData = [1 1]
      | sbobj.Groups(7).Signals(15).Name = 'state_TwoSpeed'
      | sbobj.Groups(7).Signals(15).XData = [0 100]
      | sbobj.Groups(7).Signals(15).YData = [0 0]
      | sbobj.Groups(7).Signals(16).Name = 'state_TwoSpeedIcon'
      | sbobj.Groups(7).Signals(16).XData = [0 100]
      | sbobj.Groups(7).Signals(16).YData = [0 0]
      | sbobj.Groups(7).Signals(17).Name = 'duty_TwoSpeed'
      | sbobj.Groups(7).Signals(17).XData = [0 100]
      | sbobj.Groups(7).Signals(17).YData = [0 0]
      | sbobj.Groups(7).TimeRange = [0 100]
  state_Engine : Outport  Tag=STV Outport
  state_ECT : Outport  Tag=STV Outport  Port=2
  state_HOT : Outport  Tag=STV Outport  Port=3
  state_Console : Outport  Tag=STV Outport  Port=4
  state_LoadSense : Outport  Tag=STV Outport  Port=5
  flt_HOT : Outport  Tag=STV Outport  Port=6
  Vbat : Outport  Tag=STV Outport  Port=7
  bar_Loadsense : Outport  Tag=STV Outport  Port=8
  state_System : Outport  Tag=STV Outport  Port=9
  fault : Outport  Tag=STV Outport  Port=10
  din_TwoSpeedSwitch1 : Outport  Tag=STV Outport  Port=11
  din_TwoSpeedSwitch2 : Outport  Tag=STV Outport  Port=12
  adin_TravelPressureSwitch : Outport  Tag=STV Outport  Port=13
  state_JoystickEnable : Outport  Tag=STV Outport  Port=14
  state_TwoSpeed : Outport  Tag=STV Outport  Port=15
  state_TwoSpeedIcon : Outport  Tag=STV Outport  Port=16
  duty_TwoSpeed : Outport  Tag=STV Outport  Port=17
  wires:
  FromWs/1 -> Demux/1
  Demux/1 -> state_Engine/1
  Demux/2 -> state_ECT/1
  Demux/3 -> state_HOT/1
  Demux/4 -> state_Console/1
  Demux/5 -> state_LoadSense/1
  Demux/6 -> flt_HOT/1
  Demux/7 -> Vbat/1
  Demux/8 -> bar_Loadsense/1
  Demux/9 -> state_System/1
  Demux/10 -> fault/1
  Demux/11 -> din_TwoSpeedSwitch1/1
  Demux/12 -> din_TwoSpeedSwitch2/1
  Demux/13 -> adin_TravelPressureSwitch/1
  Demux/14 -> state_JoystickEnable/1
  Demux/15 -> state_TwoSpeed/1
  Demux/16 -> state_TwoSpeedIcon/1
  Demux/17 -> duty_TwoSpeed/1

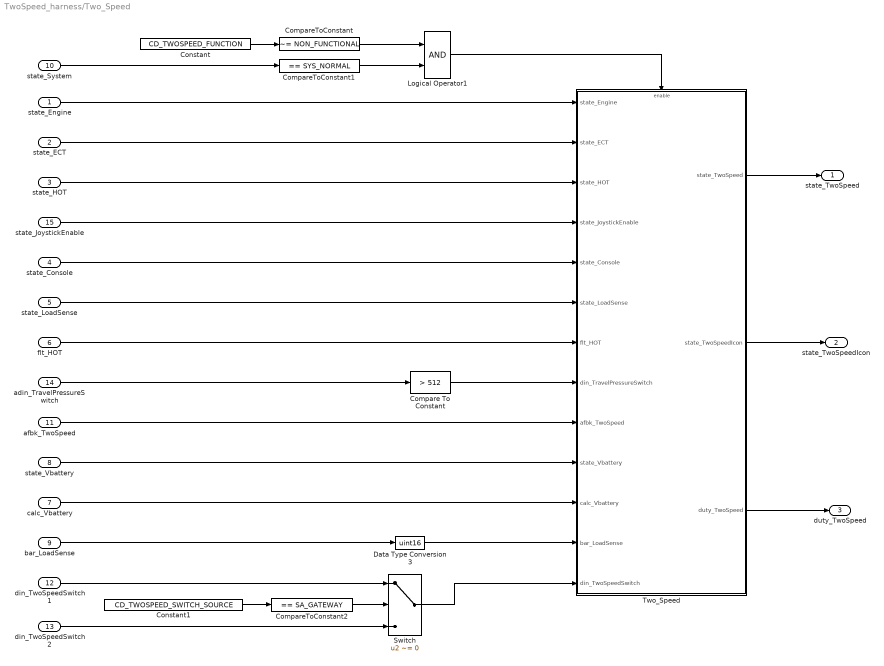
== system TwoSpeed_harness/Two_Speed ==
  state_Engine : Inport
  state_ECT : Inport  Port=2
  state_HOT : Inport  Port=3
  state_Console : Inport  Port=4
  state_LoadSense : Inport  Port=5
  flt_HOT : Inport  Port=6
  calc_Vbattery : Inport  Port=7
  state_Vbattery : Inport  Port=8
  bar_LoadSense : Inport  Port=9
  state_System : Inport  Port=10
  afbk_TwoSpeed : Inport  Port=11
  din_TwoSpeedSwitch1 : Inport  Port=12
  din_TwoSpeedSwitch2 : Inport  Port=13
  adin_TravelPressureSwitch : Inport  Port=14
  state_JoystickEnable : Inport  Port=15
  Compare To Constant : simulink/Logic and Bit Operations/Compare To Constant  SystemSampleTime=-1  relop=>  const=512  LogicOutDataTypeMode=boolean
  CompareToConstant : simulink/Logic and Bit Operations/Compare To Constant  SystemSampleTime=-1  relop=~=  const=NON_FUNCTIONAL  LogicOutDataTypeMode=boolean  ZeroCross=off
  CompareToConstant1 : simulink/Logic and Bit Operations/Compare To Constant  SystemSampleTime=-1  relop===  const=SYS_NORMAL  LogicOutDataTypeMode=boolean  ZeroCross=off
  CompareToConstant2 : simulink/Logic and Bit Operations/Compare To Constant  SystemSampleTime=-1  relop===  const=SA_GATEWAY  LogicOutDataTypeMode=boolean  ZeroCross=off
  Constant : Constant  Value=CD_TWOSPEED_FUNCTION  OutDataTypeStr=uint8
  Constant1 : Constant  Value=CD_TWOSPEED_SWITCH_SOURCE  OutDataTypeStr=uint8
  Data Type Conversion3 : DataTypeConversion  OutDataTypeStr=uint16
  Logical Operator1 : Logic  AllPortsSameDT=off  OutDataTypeStr=boolean
  Switch : Switch  Criteria=u2 ~= 0
  Two_Speed : Subsystem
  state_TwoSpeed : Outport
  state_TwoSpeedIcon : Outport  Port=2
  duty_TwoSpeed : Outport  Port=3
  wires:
  state_Engine/1 -> Two_Speed/1(state_Engine)
  state_ECT/1 -> Two_Speed/2(state_ECT)
  Constant/1 -> CompareToConstant/1
  CompareToConstant/1 -> Logical Operator1/1
  Two_Speed/1(state_TwoSpeed) -> state_TwoSpeed/1
  Two_Speed/2(state_TwoSpeedIcon) -> state_TwoSpeedIcon/1
  state_LoadSense/1 -> Two_Speed/6(state_LoadSense)
  flt_HOT/1 -> Two_Speed/7(flt_HOT)
  state_System/1 -> CompareToConstant1/1
  CompareToConstant1/1 -> Logical Operator1/2
  state_HOT/1 -> Two_Speed/3(state_HOT)
  state_JoystickEnable/1 -> Two_Speed/4(state_JoystickEnable)
  state_Console/1 -> Two_Speed/5(state_Console)
  afbk_TwoSpeed/1 -> Two_Speed/9(afbk_TwoSpeed)
  state_Vbattery/1 -> Two_Speed/10(state_Vbattery)
  calc_Vbattery/1 -> Two_Speed/11(calc_Vbattery)
  Two_Speed/3(duty_TwoSpeed) -> duty_TwoSpeed/1
  adin_TravelPressureSwitch/1 -> Compare To Constant/1
  Logical Operator1/1 -> Two_Speed/Enable
  Compare To Constant/1 -> Two_Speed/8(din_TravelPressureSwitch)
  bar_LoadSense/1 -> Data Type Conversion3/1
  Data Type Conversion3/1 -> Two_Speed/12(bar_LoadSense)
  din_TwoSpeedSwitch1/1 -> Switch/1
  din_TwoSpeedSwitch2/1 -> Switch/3
  Constant1/1 -> CompareToConstant2/1
  Switch/1 -> Two_Speed/13(din_TwoSpeedSwitch)
  CompareToConstant2/1 -> Switch/2

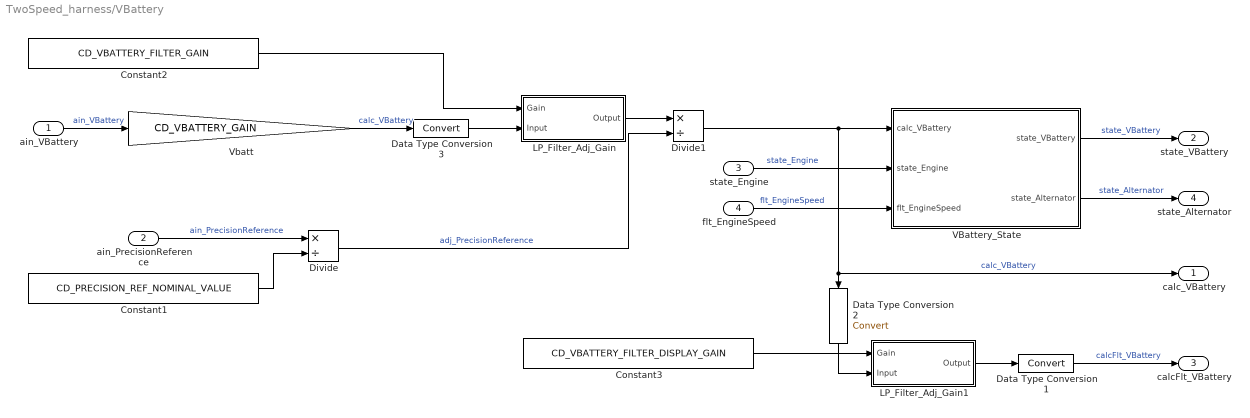
== system TwoSpeed_harness/VBattery ==
  ain_VBattery : Inport  OutDataTypeStr=uint16
  ain_PrecisionReference : Inport  Port=2  OutDataTypeStr=uint16
  state_Engine : Inport  Port=3
  flt_EngineSpeed : Inport  Port=4  OutDataTypeStr=uint16
  Constant1 : Constant  Value=CD_PRECISION_REF_NOMINAL_VALUE  OutDataTypeStr=uint16  SampleTime=srate100
  Constant2 : Constant  Value=CD_VBATTERY_FILTER_GAIN  OutDataTypeStr=uint8  SampleTime=srate100
  Constant3 : Constant  Value=CD_VBATTERY_FILTER_DISPLAY_GAIN  OutDataTypeStr=uint8  SampleTime=srate100
  Data Type Conversion1 : DataTypeConversion
  Data Type Conversion2 : DataTypeConversion
  Data Type Conversion3 : DataTypeConversion
  Divide : Product  Inputs=*/  OutDataTypeStr=fixdt(0,16,10)  RndMeth=Nearest
  Divide1 : Product  Inputs=*/  OutDataTypeStr=fixdt(0,16,8)  RndMeth=Nearest
  LP_Filter_Adj_Gain : Subsystem
  LP_Filter_Adj_Gain1 : Subsystem
  VBattery_State : Stateflow chart  TreatAsAtomicUnit=on
  Vbatt : Gain  Gain=CD_VBATTERY_GAIN  ParamDataTypeStr=fixdt(0,16,12)  OutDataTypeStr=fixdt(0,16,8)  RndMeth=Nearest  SampleTime=srate100  SaturateOnIntegerOverflow=on
  calc_VBattery : Outport
  state_VBattery : Outport  Port=2  OutDataTypeStr=uint8
  calcFlt_VBattery : Outport  Port=3  OutDataTypeStr=fixdt(0,16,8)
  state_Alternator : Outport  Port=4  OutDataTypeStr=uint8
  wires:
  ain_VBattery/1 -> Vbatt/1  "ain_VBattery"
  state_Engine/1 -> VBattery_State/2(state_Engine)  "state_Engine"
  Data Type Conversion1/1 -> calcFlt_VBattery/1  "calcFlt_VBattery"
  LP_Filter_Adj_Gain1/1(Output) -> Data Type Conversion1/1
  ain_PrecisionReference/1 -> Divide/1  "ain_PrecisionReference"
  Constant1/1 -> Divide/2
  Divide/1 -> Divide1/2  "adj_PrecisionReference"
  Vbatt/1 -> Data Type Conversion3/1  "calc_VBattery"
  Divide1/1 -> VBattery_State/1(calc_VBattery), calc_VBattery/1, Data Type Conversion2/1  "calc_VBattery"
  LP_Filter_Adj_Gain/1(Output) -> Divide1/1
  flt_EngineSpeed/1 -> VBattery_State/3(flt_EngineSpeed)  "flt_EngineSpeed"
  VBattery_State/1(state_VBattery) -> state_VBattery/1  "state_VBattery"
  VBattery_State/2(state_Alternator) -> state_Alternator/1  "state_Alternator"
  Constant2/1 -> LP_Filter_Adj_Gain/1(Gain)
  Constant3/1 -> LP_Filter_Adj_Gain1/1(Gain)
  Data Type Conversion2/1 -> LP_Filter_Adj_Gain1/2(Input)
  Data Type Conversion3/1 -> LP_Filter_Adj_Gain/2(Input)

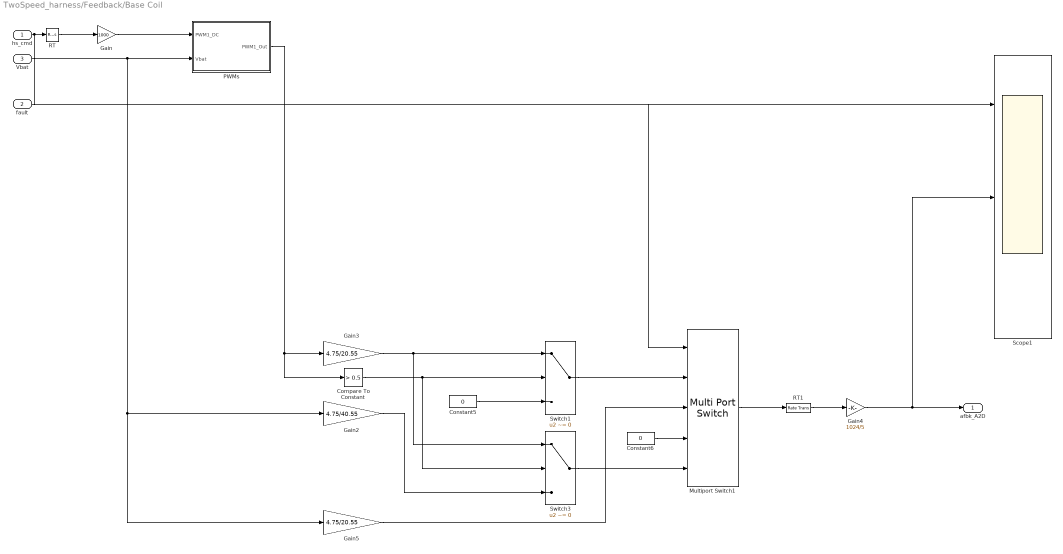
== system TwoSpeed_harness/Feedback/Base Coil ==
  hs_cmd : Inport
  fault : Inport  Port=2
  Vbat : Inport  Port=3
  Compare To Constant : simulink/Logic and Bit Operations/Compare To Constant  SystemSampleTime=-1  relop=>  const=0.5  LogicOutDataTypeMode=boolean
  Constant5 : Constant  Value=0
  Constant6 : Constant  Value=0
  Gain : Gain  Gain=1000
  Gain2 : Gain  Gain=4.75/40.55
  Gain3 : Gain  Gain=4.75/20.55
  Gain4 : Gain  Gain=1024/5  OutDataTypeStr=uint16
  Gain5 : Gain  Gain=4.75/20.55
  Multiport Switch1 : MultiPortSwitch  DataPortOrder=Zero-based contiguous  Inputs=4  zeroidx=on
  PWMs : Subsystem
  RT : RateTransition  OutPortSampleTime=0
  RT1 : RateTransition  OutPortSampleTime=.01
  Scope1 : Scope  NumInputPorts=3
      settings: TimeRange=50  YMin=0~0~0  YMax=0.3~1~1.25  SaveName=ScopeData2  DataFormat=Array
  Switch1 : Switch  Criteria=u2 ~= 0
  Switch3 : Switch  Criteria=u2 ~= 0
  afbk_A2D : Outport
  wires:
  Vbat/1 -> PWMs/2(Vbat), Gain5/1, Gain2/1
  PWMs/1(PWM1_Out) -> Gain3/1, Compare To Constant/1
  Gain/1 -> PWMs/1(PWM1_DC)
  hs_cmd/1 -> RT/1, Scope1/1
  RT/1 -> Gain/1
  fault/1 -> Multiport Switch1/1
  Compare To Constant/1 -> Switch1/2, Switch3/2
  Gain3/1 -> Switch1/1, Switch3/1
  Switch1/1 -> Multiport Switch1/2
  Constant5/1 -> Switch1/3
  Gain2/1 -> Switch3/3
  Multiport Switch1/1 -> RT1/1
  Gain4/1 -> afbk_A2D/1, Scope1/2
  Gain5/1 -> Multiport Switch1/3
  Constant6/1 -> Multiport Switch1/4
  RT1/1 -> Gain4/1
  Switch3/1 -> Multiport Switch1/5

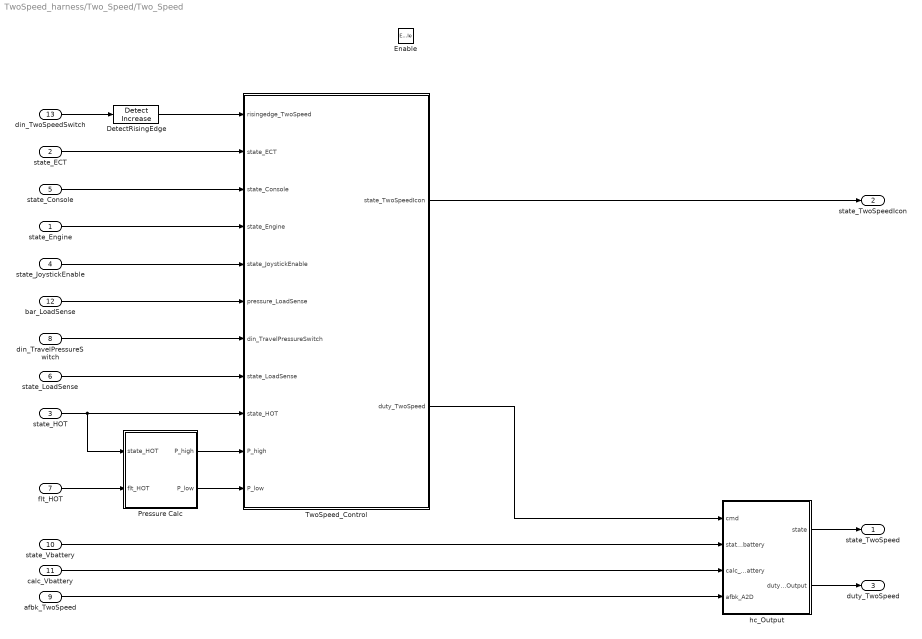
== system TwoSpeed_harness/Two_Speed/Two_Speed ==
  state_Engine : Inport
  state_ECT : Inport  Port=2
  state_HOT : Inport  Port=3
  state_JoystickEnable : Inport  Port=4
  state_Console : Inport  Port=5
  state_LoadSense : Inport  Port=6
  flt_HOT : Inport  Port=7
  din_TravelPressureSwitch : Inport  Port=8
  afbk_TwoSpeed : Inport  Port=9
  state_Vbattery : Inport  Port=10
  calc_Vbattery : Inport  Port=11
  bar_LoadSense : Inport  Port=12
  din_TwoSpeedSwitch : Inport  Port=13
  Enable : EnablePort  StatesWhenEnabling=reset  PropagateVarSize=During execution
  DetectRisingEdge : simulink/Logic and Bit Operations/Detect Increase  SystemSampleTime=-1  vinit=0.0
  Pressure Calc : Subsystem
  TwoSpeed_Control : Stateflow chart  TreatAsAtomicUnit=on
  hc_Output : Subsystem  AncestorBlock=MX_Library/output_single_OpenLoop  TreatAsAtomicUnit=on  RTWFileName=mod_Library  mask{FUNCTION=CD_TWOSPEED_FUNCTION, AFBK_GAIN=CD_TWOSPEED_AFBK_GAIN, OPEN_DB_CNT=CD_TWOSPEED_DEBOUNCE_OPEN_CIRCUIT, STB_DB_CNT=CD_TWOSPEED_DEBOUNCE_SHORT_TO_BATTERY, STG_DB_CNT=CD_TWOSPEED_DEBOUNCE_SHORT_TO_GROUND}
      mask prompts: FUNCTION "Functional:"; AFBK_GAIN "Analog Feedback Gain: -storage: fi(0,16,8)"; OPEN_DB_CNT "Debounce Open Circuit: -storage: uint(16)"; STB_DB_CNT "Debounce STB: -storage: uint(16)"; STG_DB_CNT "Debounce STG: -storage: uint(16)"
      settings: RTWFcnNameOpts=Use subsystem name  RTWFileNameOpts=User specified
  state_TwoSpeed : Outport  OutputWhenDisabled=reset  InitialOutput=[0]
  state_TwoSpeedIcon : Outport  Port=2  OutputWhenDisabled=reset  InitialOutput=[0]
  duty_TwoSpeed : Outport  Port=3  OutputWhenDisabled=reset  InitialOutput=[0]
  wires:
  din_TwoSpeedSwitch/1 -> DetectRisingEdge/1
  state_ECT/1 -> TwoSpeed_Control/2(state_ECT)
  state_HOT/1 -> TwoSpeed_Control/9(state_HOT), Pressure Calc/1(state_HOT)
  state_Console/1 -> TwoSpeed_Control/3(state_Console)
  state_Engine/1 -> TwoSpeed_Control/4(state_Engine)
  state_JoystickEnable/1 -> TwoSpeed_Control/5(state_JoystickEnable)
  DetectRisingEdge/1 -> TwoSpeed_Control/1(risingedge_TwoSpeed)
  din_TravelPressureSwitch/1 -> TwoSpeed_Control/7(din_TravelPressureSwitch)
  bar_LoadSense/1 -> TwoSpeed_Control/6(pressure_LoadSense)
  state_LoadSense/1 -> TwoSpeed_Control/8(state_LoadSense)
  Pressure Calc/1(P_high) -> TwoSpeed_Control/10(P_high)
  Pressure Calc/2(P_low) -> TwoSpeed_Control/11(P_low)
  flt_HOT/1 -> Pressure Calc/2(flt_HOT)
  TwoSpeed_Control/1(state_TwoSpeedIcon) -> state_TwoSpeedIcon/1
  hc_Output/1(state) -> state_TwoSpeed/1
  hc_Output/2(duty_Output) -> duty_TwoSpeed/1
  TwoSpeed_Control/2(duty_TwoSpeed) -> hc_Output/1(cmd)
  afbk_TwoSpeed/1 -> hc_Output/4(afbk_A2D)
  state_Vbattery/1 -> hc_Output/2(state_Vbattery)
  calc_Vbattery/1 -> hc_Output/3(calc_VBattery)

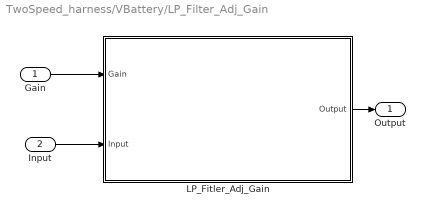
== system TwoSpeed_harness/VBattery/LP_Filter_Adj_Gain ==
  Gain : Inport
  Input : Inport  Port=2
  LP_Fitler_Adj_Gain : Stateflow chart  TreatAsAtomicUnit=on
  Output : Outport
  wires:
  LP_Fitler_Adj_Gain/1(Output) -> Output/1
  Input/1 -> LP_Fitler_Adj_Gain/2(Input)
  Gain/1 -> LP_Fitler_Adj_Gain/1(Gain)

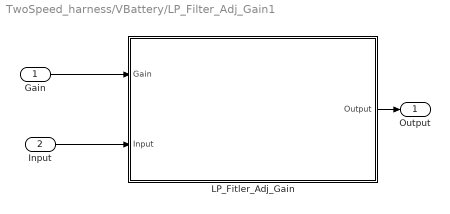
== system TwoSpeed_harness/VBattery/LP_Filter_Adj_Gain1 ==
  Gain : Inport
  Input : Inport  Port=2
  LP_Fitler_Adj_Gain : Stateflow chart  TreatAsAtomicUnit=on
  Output : Outport
  wires:
  LP_Fitler_Adj_Gain/1(Output) -> Output/1
  Input/1 -> LP_Fitler_Adj_Gain/2(Input)
  Gain/1 -> LP_Fitler_Adj_Gain/1(Gain)

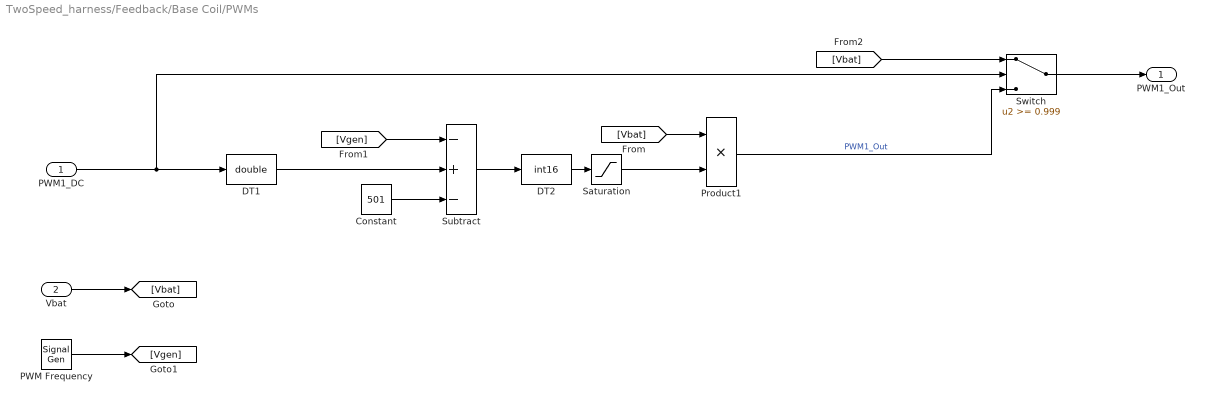
== system TwoSpeed_harness/Feedback/Base Coil/PWMs ==
  PWM1_DC : Inport
  Vbat : Inport  Port=2  OutDataTypeStr=double
  Constant : Constant  Value=501
  DT1 : DataTypeConversion  OutDataTypeStr=double  SampleTime=0
  DT2 : DataTypeConversion  OutDataTypeStr=int16  SampleTime=0
  PWM Frequency : SignalGenerator  WaveForm=sawtooth  Amplitude=500  Frequency=100
  Product1 : Product  OutDataTypeStr=double  RndMeth=Zero
  Saturation : Saturate  UpperLimit=1  LowerLimit=0
  Subtract : Sum  Inputs=-+-
  Switch : Switch  Threshold=0.999
  PWM1_Out : Outport
  wires:
  Subtract/1 -> DT2/1
  DT1/1 -> Subtract/2
  Constant/1 -> Subtract/3
  DT2/1 -> Saturation/1
  Vbat/1 -> [Vbat]
  [Vbat] -> Product1/1
  PWM Frequency/1 -> [Vgen]
  [Vgen] -> Subtract/1
  PWM1_DC/1 -> DT1/1, Switch/2
  Saturation/1 -> Product1/2
  Product1/1 -> Switch/3  "PWM1_Out"
  Switch/1 -> PWM1_Out/1
  [Vbat] -> Switch/1

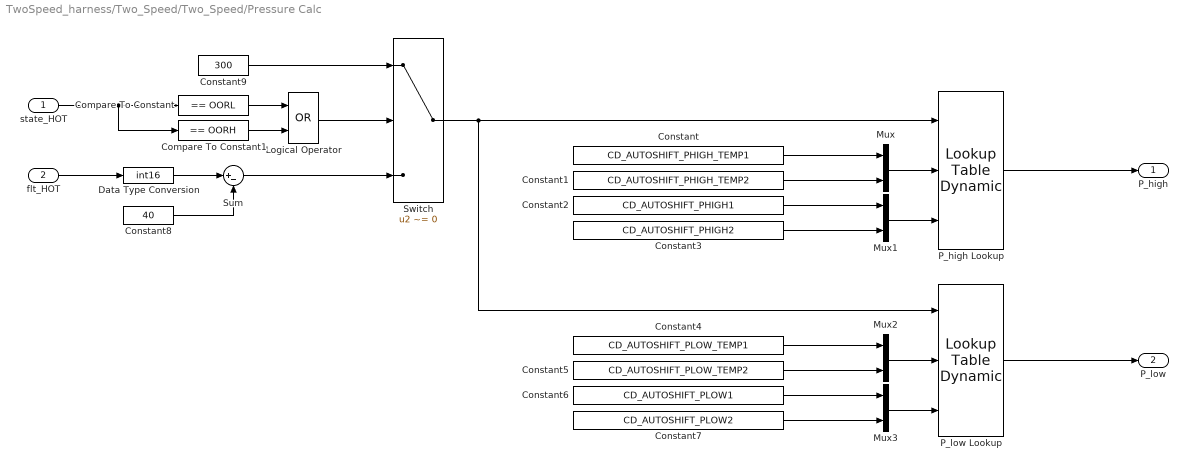
== system TwoSpeed_harness/Two_Speed/Two_Speed/Pressure Calc ==
  state_HOT : Inport
  flt_HOT : Inport  Port=2
  Compare To Constant : simulink/Logic and Bit Operations/Compare To Constant  SystemSampleTime=-1  relop===  const=OORL  LogicOutDataTypeMode=boolean
  Compare To Constant1 : simulink/Logic and Bit Operations/Compare To Constant  SystemSampleTime=-1  relop===  const=OORH  LogicOutDataTypeMode=boolean
  Constant : Constant  Value=CD_AUTOSHIFT_PHIGH_TEMP1  OutDataTypeStr=int16
  Constant1 : Constant  Value=CD_AUTOSHIFT_PHIGH_TEMP2  OutDataTypeStr=int16
  Constant2 : Constant  Value=CD_AUTOSHIFT_PHIGH1  OutDataTypeStr=uint16
  Constant3 : Constant  Value=CD_AUTOSHIFT_PHIGH2  OutDataTypeStr=uint16
  Constant4 : Constant  Value=CD_AUTOSHIFT_PLOW_TEMP1  OutDataTypeStr=int16
  Constant5 : Constant  Value=CD_AUTOSHIFT_PLOW_TEMP2  OutDataTypeStr=int16
  Constant6 : Constant  Value=CD_AUTOSHIFT_PLOW1  OutDataTypeStr=uint16
  Constant7 : Constant  Value=CD_AUTOSHIFT_PLOW2  OutDataTypeStr=uint16
  Constant8 : Constant  Value=40  OutDataTypeStr=uint8
  Constant9 : Constant  Value=300  OutDataTypeStr=int16
  Data Type Conversion : DataTypeConversion  OutDataTypeStr=int16
  Logical Operator : Logic  Operator=OR  AllPortsSameDT=off  OutDataTypeStr=boolean
  Mux{,1..3} (4 alike) : Mux  Inputs=2
  P_high Lookup : simulink/Lookup Tables/Lookup Table Dynamic  LookUpMeth=Interpolation-Use End Values  OutDataTypeStr=fixdt('uint16')  OutputDataTypeScalingMode=Specify via dialog  OutDataType=fixdt('uint16')  OutScaling=[]  DoSatur=off
  P_low Lookup : simulink/Lookup Tables/Lookup Table Dynamic  LookUpMeth=Interpolation-Use End Values  OutDataTypeStr=fixdt('uint16')  OutputDataTypeScalingMode=Specify via dialog  OutDataType=fixdt('uint16')  OutScaling=[]  DoSatur=off
  Sum : Sum  Inputs=|+-
  Switch : Switch  Criteria=u2 ~= 0
  P_high : Outport
  P_low : Outport  Port=2
  wires:
  flt_HOT/1 -> Data Type Conversion/1
  P_high Lookup/1 -> P_high/1
  P_low Lookup/1 -> P_low/1
  Constant/1 -> Mux/1
  Constant1/1 -> Mux/2
  Constant2/1 -> Mux1/1
  Constant3/1 -> Mux1/2
  Mux/1 -> P_high Lookup/2
  Mux1/1 -> P_high Lookup/3
  Constant4/1 -> Mux2/1
  Constant5/1 -> Mux2/2
  Constant6/1 -> Mux3/1
  Constant7/1 -> Mux3/2
  Mux2/1 -> P_low Lookup/2
  Mux3/1 -> P_low Lookup/3
  Data Type Conversion/1 -> Sum/1
  Constant8/1 -> Sum/2
  Compare To Constant/1 -> Logical Operator/1
  Compare To Constant1/1 -> Logical Operator/2
  state_HOT/1 -> Compare To Constant/1, Compare To Constant1/1
  Sum/1 -> Switch/3
  Switch/1 -> P_high Lookup/1, P_low Lookup/1
  Logical Operator/1 -> Switch/2
  Constant9/1 -> Switch/1

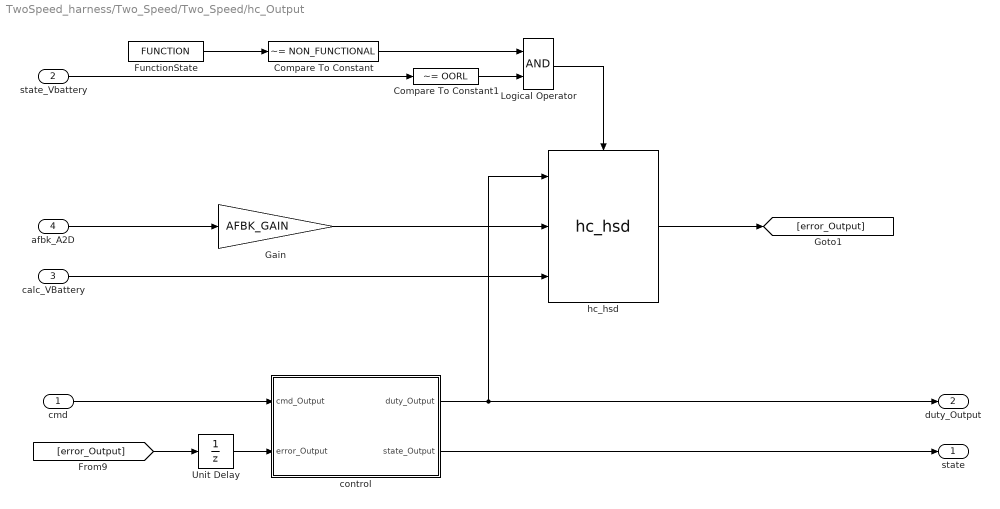
== system TwoSpeed_harness/Two_Speed/Two_Speed/hc_Output ==
  cmd : Inport
  state_Vbattery : Inport  Port=2
  calc_VBattery : Inport  Port=3
  afbk_A2D : Inport  Port=4  OutDataTypeStr=uint16
  Compare To Constant : simulink/Logic and Bit Operations/Compare To Constant  SystemSampleTime=-1  relop=~=  const=NON_FUNCTIONAL  LogicOutDataTypeMode=boolean  ZeroCross=off
  Compare To Constant1 : simulink/Logic and Bit Operations/Compare To Constant  SystemSampleTime=-1  relop=~=  const=OORL  LogicOutDataTypeMode=boolean  ZeroCross=off
  FunctionState : Constant  Value=FUNCTION  OutDataTypeStr=uint8  SampleTime=-1
  Gain : Gain  Gain=AFBK_GAIN  ParamDataTypeStr=fixdt(0,16,8)  OutDataTypeStr=fixdt(0,16,8)  RndMeth=Zero  SaturateOnIntegerOverflow=on
  Logical Operator : Logic  AllPortsSameDT=off  OutDataTypeStr=boolean
  Unit Delay : UnitDelay  SampleTime=-1
  control : Stateflow chart
  hc_hsd : MX_Library/hc_hsd  SystemSampleTime=-1  STB_DB_CNT=STB_DB_CNT  STG_DB_CNT=STG_DB_CNT  OPEN_DB_CNT=OPEN_DB_CNT
  state : Outport
  duty_Output : Outport  Port=2
  wires:
  Unit Delay/1 -> control/2(error_Output)
  control/2(state_Output) -> state/1
  control/1(duty_Output) -> hc_hsd/1, duty_Output/1
  [error_Output] -> Unit Delay/1
  hc_hsd/1 -> [error_Output]
  cmd/1 -> control/1(cmd_Output)
  state_Vbattery/1 -> Compare To Constant1/1
  FunctionState/1 -> Compare To Constant/1
  Compare To Constant/1 -> Logical Operator/1
  calc_VBattery/1 -> hc_hsd/3
  afbk_A2D/1 -> Gain/1
  Gain/1 -> hc_hsd/2
  Compare To Constant1/1 -> Logical Operator/2
  Logical Operator/1 -> hc_hsd/Enable

== stateflow chart VBattery/LP_Filter_Adj_Gain/LP_Fitler_Adj_Gain ==
  state INITIAL
    en:Output = Input;
  state LP_FILTER
    du:Output = Output + ((Input - Output)/(1 << Gain));
  (default) -> INITIAL
  INITIAL -> LP_FILTER
  data: Gain input uint8; Input input fixdt(1,16,8); Output output fixdt(1,32,16)

== stateflow chart VBattery/VBattery_State ==
  state NON_FUNCTIONAL
    en:state_VBattery = NORMAL;
    en:state_Alternator = NORMAL;
  state NORMAL
    state NORMAL
      state NORMAL
        en:state_VBattery = NORMAL;
        en:state_Alternator = NORMAL;
      state DEBOUNCE
        en:debounceCount = 0;
        du:debounceCount++;
      (default) -> NORMAL.NORMAL.DEBOUNCE
      NORMAL.NORMAL.DEBOUNCE -> NORMAL.NORMAL.NORMAL : [(debounceCount >= CD_VBATTERY_DEBOUNCE_NORMAL)...
          | || ((state_VBattery == NORMAL) && (state_Alternator == NORMAL))]
    state HIGH
      state HIGH
        en:state_VBattery = HIGH;
        en:state_Alternator = NORMAL;
      state DEBOUNCE
        en:debounceCount = 0;
        du:debounceCount++;
      NORMAL.HIGH.DEBOUNCE -> NORMAL.HIGH.HIGH : [(debounceCount >= CD_VBATTERY_DEBOUNCE_HIGH)...
          | || (state_VBattery == HIGH)]
      (default) -> NORMAL.HIGH.DEBOUNCE
    state EXTREMELY_LOW
      state DEBOUNCE
        en:debounceCount = 0;
        du:debounceCount++;
      state EXTREMELY_LOW
        en:state_VBattery = EXTREMELY_LOW;
        en:state_Alternator = NORMAL;
      NORMAL.EXTREMELY_LOW.DEBOUNCE -> NORMAL.EXTREMELY_LOW.EXTREMELY_LOW : [(debounceCount >= CD_VBATTERY_DEBOUNCE_EXTREMELY_LOW)...
          | || (state_VBattery == EXTREMELY_LOW)]
      (default) -> NORMAL.EXTREMELY_LOW.DEBOUNCE
    state LOW
      state LOW
        en:state_VBattery = LOW;
        en:state_Alternator = NORMAL;
      state DEBOUNCE
        en:debounceCount = 0;
        du:debounceCount++;
      NORMAL.LOW.DEBOUNCE -> NORMAL.LOW.LOW : [(debounceCount >= CD_VBATTERY_DEBOUNCE_LOW)...
          | || (state_VBattery == LOW)]
      (default) -> NORMAL.LOW.DEBOUNCE
    state EXTREMELY_HIGH
      state DEBOUNCE
        en:debounceCount = 0;
        du:debounceCount++;
      state EXTREMELY_HIGH
        en:state_VBattery = EXTREMELY_HIGH;
        en:state_Alternator = NORMAL;
      NORMAL.EXTREMELY_HIGH.DEBOUNCE -> NORMAL.EXTREMELY_HIGH.EXTREMELY_HIGH : [(debounceCount >= CD_VBATTERY_DEBOUNCE_EXTREMELY_HIGH)...
          | || (state_VBattery == EXTREMELY_HIGH)]
      (default) -> NORMAL.EXTREMELY_HIGH.DEBOUNCE
    state ALTERNATOR_LOW
      state DEBOUNCE
        en:debounceCount = 0;
        du:debounceCount++;
      state LOW
        en:state_Alternator = LOW;
        en:state_VBattery = NORMAL;
      (default) -> NORMAL.ALTERNATOR_LOW.DEBOUNCE
      NORMAL.ALTERNATOR_LOW.DEBOUNCE -> NORMAL.ALTERNATOR_LOW.LOW : [(debounceCount >= CD_ALTERNATOR_DEBOUNCE_LOW)]
    state ALTERNATOR_HIGH
      state DEBOUNCE
        en:debounceCount = 0;
        du:debounceCount++;
      state HIGH
        en:state_Alternator = HIGH;
        en:state_VBattery = NORMAL;
      (default) -> NORMAL.ALTERNATOR_HIGH.DEBOUNCE
      NORMAL.ALTERNATOR_HIGH.DEBOUNCE -> NORMAL.ALTERNATOR_HIGH.HIGH : [(debounceCount >= CD_ALTERNATOR_DEBOUNCE_HIGH)]
    NORMAL.EXTREMELY_HIGH -> NORMAL.HIGH [order 2] : [(calc_VBattery < (CD_VBATTERY_EXTREMELY_HIGH - CD_VOLTAGE_HYSTERESIS))...
        | && ((CD_ALTERNATOR_FUNCTION ==NON_FUNCTIONAL)...
        |   || (flt_EngineSpeed < CD_ALTERNATOR_ALARM_ENGINE_SPEED))]
    NORMAL.HIGH -> NORMAL.EXTREMELY_HIGH [order 1] : [(calc_VBattery >= CD_VBATTERY_EXTREMELY_HIGH)]
    (default) -> NORMAL.NORMAL
    NORMAL.HIGH -> NORMAL.NORMAL [order 2] : [(calc_VBattery < (CD_VBATTERY_HIGH - CD_VOLTAGE_HYSTERESIS))]
    NORMAL.NORMAL -> NORMAL.HIGH [order 3] : [(calc_VBattery >= CD_VBATTERY_HIGH)...
        | && ((CD_ALTERNATOR_FUNCTION ==NON_FUNCTIONAL)...
        |    ||  (flt_EngineSpeed < CD_ALTERNATOR_ALARM_ENGINE_SPEED))]
    NORMAL.NORMAL -> NORMAL.LOW [order 4] : [(calc_VBattery <= CD_VBATTERY_LOW)...
        | && ((CD_ALTERNATOR_FUNCTION == NON_FUNCTIONAL)...
        |   ||  (flt_EngineSpeed < CD_ALTERNATOR_ALARM_ENGINE_SPEED))]
    NORMAL.LOW -> NORMAL.NORMAL [order 1] : [(calc_VBattery > (CD_VBATTERY_LOW + CD_VOLTAGE_HYSTERESIS))...
        | && (state_Engine != ENGINE_CRANKING)]
    NORMAL.LOW -> NORMAL.EXTREMELY_LOW [order 2] : [(calc_VBattery <= CD_VBATTERY_EXTREMELY_LOW)]
    NORMAL.EXTREMELY_LOW -> NORMAL.LOW [order 2] : [(calc_VBattery > (CD_VBATTERY_EXTREMELY_LOW + CD_VOLTAGE_HYSTERESIS))...
        | && (state_Engine != ENGINE_CRANKING)...
        | && ((CD_ALTERNATOR_FUNCTION == NON_FUNCTIONAL)...
        |   ||  (flt_EngineSpeed < CD_ALTERNATOR_ALARM_ENGINE_SPEED))]
    NORMAL.NORMAL -> ALTERNATOR_LOW [order 1] : [(CD_ALTERNATOR_FUNCTION != NON_FUNCTIONAL)...
        | && (calc_VBattery <= CD_ALTERNATOR_LOW)...
        | && (flt_EngineSpeed >= CD_ALTERNATOR_ALARM_ENGINE_SPEED)]
    ALTERNATOR_LOW -> NORMAL.NORMAL [order 1] : [(calc_VBattery > (CD_ALTERNATOR_LOW + CD_VOLTAGE_HYSTERESIS))...
        | || (flt_EngineSpeed < CD_ALTERNATOR_ALARM_ENGINE_SPEED)]
    NORMAL.NORMAL -> ALTERNATOR_HIGH [order 2] : [(CD_ALTERNATOR_FUNCTION != NON_FUNCTIONAL)...
        | && (calc_VBattery >= CD_ALTERNATOR_HIGH)...
        | && (flt_EngineSpeed >= CD_ALTERNATOR_ALARM_ENGINE_SPEED)]
    ALTERNATOR_HIGH -> NORMAL.NORMAL [order 1] : [(calc_VBattery < (CD_ALTERNATOR_HIGH - CD_VOLTAGE_HYSTERESIS))...
        | || (flt_EngineSpeed < CD_ALTERNATOR_ALARM_ENGINE_SPEED)]
    NORMAL.EXTREMELY_LOW -> ALTERNATOR_LOW [order 1] : [(calc_VBattery > (CD_VBATTERY_EXTREMELY_LOW + CD_VOLTAGE_HYSTERESIS))...
        | && ((CD_ALTERNATOR_FUNCTION != NON_FUNCTIONAL) && (flt_EngineSpeed >= CD_ALTERNATOR_ALARM_ENGINE_SPEED))]
    ALTERNATOR_LOW -> NORMAL.EXTREMELY_LOW [order 2] : [(calc_VBattery <= CD_VBATTERY_EXTREMELY_LOW)]
    ALTERNATOR_HIGH -> NORMAL.EXTREMELY_HIGH [order 2] : [(calc_VBattery >= CD_VBATTERY_EXTREMELY_HIGH)]
    NORMAL.EXTREMELY_HIGH -> ALTERNATOR_HIGH [order 1] : [(calc_VBattery < (CD_VBATTERY_EXTREMELY_HIGH - CD_VOLTAGE_HYSTERESIS))...
        | && ((CD_ALTERNATOR_FUNCTION != NON_FUNCTIONAL) && (flt_EngineSpeed >= CD_ALTERNATOR_ALARM_ENGINE_SPEED))]
  state OORL
    state DEBOUNCE_OORL
      en:debounceCount = 0;
      du:debounceCount++;
    state OORL
      en:state_VBattery = OORL;
      en:state_Alternator = NORMAL;
    DEBOUNCE_OORL -> OORL.OORL : [(debounceCount >= CD_VBATTERY_DEBOUNCE_OORL)...
        | || (state_VBattery == OORL)]
    (default) -> DEBOUNCE_OORL
  (default) -> NON_FUNCTIONAL
  NORMAL -> OORL : [(calc_VBattery <= CD_VBATTERY_OORL)]
  OORL -> NORMAL : [(state_Engine != ENGINE_CRANKING)...
      | && (calc_VBattery > (CD_VBATTERY_OORL + CD_VOLTAGE_HYSTERESIS))]
  NON_FUNCTIONAL -> NORMAL : [(CD_VBATTERY_FUNCTION != NON_FUNCTIONAL)]
  data: state_VBattery output uint8; calc_VBattery input fixdt(0,16,8); debounceCount local uint16 =0; CD_VBATTERY_DEBOUNCE_EXTREMELY_LOW parameter uint16; CD_VBATTERY_DEBOUNCE_HIGH parameter uint16; CD_VBATTERY_DEBOUNCE_LOW parameter uint16; CD_VBATTERY_DEBOUNCE_NORMAL parameter uint16; CD_VBATTERY_DEBOUNCE_OORL parameter uint16; CD_VBATTERY_EXTREMELY_LOW parameter uint16; CD_VBATTERY_FUNCTION parameter uint8; CD_VBATTERY_HIGH parameter uint8; CD_VBATTERY_LOW parameter uint8; CD_VBATTERY_OORL parameter uint8; state_Engine input uint8; CD_VBATTERY_EXTREMELY_HIGH parameter uint8; CD_VBATTERY_DEBOUNCE_EXTREMELY_HIGH parameter uint16; HIGH parameter uint8 =10; OORL parameter uint8 =22; LOW parameter uint8 =9; NORMAL parameter uint8 =8; EXTREMELY_LOW parameter uint8 =14; EXTREMELY_HIGH parameter uint8 =11; ENGINE_CRANKING parameter uint8 =2; NON_FUNCTIONAL parameter uint8 =255; CD_VOLTAGE_HYSTERESIS parameter fixdt(0,8,4); CD_ALTERNATOR_FUNCTION parameter uint8; CD_ALTERNATOR_HIGH parameter uint8; CD_ALTERNATOR_LOW parameter uint8; state_Alternator output uint8; CD_ALTERNATOR_ALARM_ENGINE_SPEED parameter uint16; flt_EngineSpeed input uint16; CD_ALTERNATOR_DEBOUNCE_HIGH parameter uint16; CD_ALTERNATOR_DEBOUNCE_LOW parameter uint16

== stateflow chart Two_Speed/Two_Speed/hc_Output/control ==
  state ERROR
    en:duty_Output = INACTIVE;
    en:state_Output = error_Output;
  state FUNCTIONAL
    en:
    duty_Output = cmd_Output;
    du:
    duty_Output = cmd_Output;
    state ACTIVE
      en:
      state_Output = ACTIVE;
    state INACTIVE
      en:
      state_Output = INACTIVE;
    INACTIVE -> ACTIVE : [cmd_Output != INACTIVE]
    (default) -> INACTIVE
    ACTIVE -> INACTIVE : [cmd_Output == INACTIVE]
  FUNCTIONAL -> ERROR : [(error_Output != NORMAL)]
  ERROR -> FUNCTIONAL : [(error_Output == NORMAL)]
  (default) -> FUNCTIONAL
  data: duty_Output output fixdt(0,16,16); state_Output output uint8; cmd_Output input fixdt(0,16,16); error_Output input uint8; INACTIVE parameter uint8 =0; ACTIVE parameter uint8 =1; NORMAL parameter uint8

== stateflow chart Two_Speed/Two_Speed/TwoSpeed_Control ==
  state Control [parallel]
    settings: executionOrder=1
    state AutoShift
      state Inactive
        en:
        cmd_TwoSpeed = INACTIVE;
        state_TwoSpeedIcon = INACTIVE;
      state Active
        state Autoshift_Inactive
          en:
          cmd_TwoSpeed = LOW;
          state_TwoSpeedIcon = INACTIVE;
        state Autoshift_Active
          en:
          state_TwoSpeedIcon = ACTIVE;
          state Low_Travel
            en:
            cmd_TwoSpeed = LOW;
          state Delay
          state Low_No_Travel
            en:
            cmd_TwoSpeed = LOW;
          state High
            en:
            cmd_TwoSpeed = HIGH;
          Delay -> Control.AutoShift.Active.Autoshift_Active.High [order 1] : [after(CD_AUTOSHIFT_TRAVEL_DELAY, tick)]
          Delay -> Low_No_Travel [order 2] : [din_TravelPressureSwitch == INACTIVE]
          Low_Travel -> Control.AutoShift.Active.Autoshift_Active.High [order 2] : [pressure_LoadSense < P_low...
              | || state_LoadSense != NORMAL]
          Low_Travel -> Low_No_Travel [order 1] : [din_TravelPressureSwitch == INACTIVE]
          (junction 149) -> Delay [order 1] : [CD_AUTOSHIFT_TRAVEL_DELAY > 0]
          (junction 148) -> Control.AutoShift.Active.Autoshift_Active.High
          (junction 149) -> (junction 148) [order 2]
          Control.AutoShift.Active.Autoshift_Active.High -> Low_No_Travel [order 2] : [din_TravelPressureSwitch == INACTIVE]
          (default) -> Low_No_Travel
          Low_No_Travel -> (junction 149) : [din_TravelPressureSwitch == ACTIVE]
          Control.AutoShift.Active.Autoshift_Active.High -> Low_Travel [order 1] : [pressure_LoadSense > P_high...
              | && state_LoadSense == NORMAL]
        (default) -> Autoshift_Inactive
        Autoshift_Active -> Autoshift_Inactive : [risingedge_TwoSpeed]
        Autoshift_Inactive -> Autoshift_Active : [risingedge_TwoSpeed]
      (default) -> Control.AutoShift.Inactive
      Control.AutoShift.Active -> Control.AutoShift.Inactive : [state_Console != ACTIVE...
          | || state_HOT == HIGH...
          | || state_HOT == EXTREMELY_HIGH...
          | || state_ECT == HIGH...
          | || state_ECT == EXTREMELY_HIGH]
      Control.AutoShift.Inactive -> Control.AutoShift.Active : [state_Console == ACTIVE...
          | && state_HOT != HIGH...
          | && state_HOT != EXTREMELY_HIGH...
          | && state_ECT != HIGH...
          | && state_ECT != EXTREMELY_HIGH]
    state Normal
      state Inactive
        en:
        cmd_TwoSpeed = INACTIVE;
        state_TwoSpeedIcon = INACTIVE;
      state Active
        state High
          en:
          cmd_TwoSpeed = HIGH;
          state_TwoSpeedIcon = ACTIVE;
        state Low
          en:
          cmd_TwoSpeed = LOW;
          state_TwoSpeedIcon = INACTIVE;
        (default) -> Control.Normal.Active.Low
        Control.Normal.Active.Low -> Control.Normal.Active.High : [risingedge_TwoSpeed]
        Control.Normal.Active.High -> Control.Normal.Active.Low : [risingedge_TwoSpeed]
      Control.Normal.Active -> Control.Normal.Inactive : [state_Console != ACTIVE...
          | || state_HOT == HIGH...
          | || state_HOT == EXTREMELY_HIGH...
          | || state_ECT == HIGH...
          | || state_ECT == EXTREMELY_HIGH]
      Control.Normal.Inactive -> Control.Normal.Active : [state_Console == ACTIVE...
          | && state_HOT != HIGH...
          | && state_HOT != EXTREMELY_HIGH...
          | && state_ECT != HIGH...
          | && state_ECT != EXTREMELY_HIGH]
      (default) -> Control.Normal.Inactive
    state NonFunctional
      en:
      cmd_TwoSpeed = INACTIVE;
      state_TwoSpeedIcon = INACTIVE;
    (junction 150) -> Normal [order 2]
    (junction 150) -> AutoShift [order 1] : [CD_AUTOSHIFT_FUNCTION != NON_FUNCTIONAL]
    (default) -> NonFunctional
    NonFunctional -> (junction 150)
  state Two_Speed_Command [parallel]
    settings: executionOrder=2
    state High
      en:
      duty_TwoSpeed = FULL_ON;
    state Low
      en:
      duty_TwoSpeed = INACTIVE;
    (default) -> Two_Speed_Command.Low
    Two_Speed_Command.High -> Two_Speed_Command.Low : [cmd_TwoSpeed != HIGH...
        | || state_Engine == ENGINE_CRANKING...
        | || state_JoystickEnable != ACTIVE]
    Two_Speed_Command.Low -> Two_Speed_Command.High : [cmd_TwoSpeed == HIGH...
        | && state_Engine != ENGINE_CRANKING...
        | && state_JoystickEnable == ACTIVE]
  data: risingedge_TwoSpeed input uint8; cmd_TwoSpeed local uint8; FULL_ON parameter fixdt(0,16,16); EXTREMELY_HIGH parameter uint8; state_ECT input uint8; HIGH parameter uint8; INACTIVE parameter uint8; LOW parameter uint8; state_Console input uint8; state_Engine input uint8; ENGINE_CRANKING parameter uint8; state_JoystickEnable input uint8; NORMAL parameter uint8; CD_TWOSPEED_FUNCTION parameter uint8; CD_AUTOSHIFT_FUNCTION parameter uint8; pressure_LoadSense input uint16; din_TravelPressureSwitch input boolean; state_TwoSpeedIcon output uint8; duty_TwoSpeed output fixdt(0,16,16); CD_AUTOSHIFT_TRAVEL_DELAY parameter uint8; NON_FUNCTIONAL parameter uint8; state_LoadSense input uint8; state_HOT input uint8; P_high input uint16; P_low input uint16; ACTIVE parameter uint8

== stateflow chart VBattery/LP_Filter_Adj_Gain1/LP_Fitler_Adj_Gain ==
  state INITIAL
    en:Output = Input;
  state LP_FILTER
    du:Output = Output + ((Input - Output)/(1 << Gain));
  (default) -> INITIAL
  INITIAL -> LP_FILTER
  data: Gain input uint8; Input input fixdt(1,16,8); Output output fixdt(1,32,16)
